simulink library "ammclib_bam_S32K3xx"  (R2016a)
(part 40 of 50)

      |       SampleTime=SampleTime_1;
      |       if isnan(SampleTime)
      |         hintText.Prompt='Note: Implementation parameters cannot be calculated yet because the block''s inherited sample time is unknown. Simulink will update the sample time when you run the simulation.';
      |       else
      |         hintText.Prompt='Caution: Implementation parameters depend on inherited sample time. Make sure that the sample time of the block''s inputs corresponds to the sampling period in the target application.';
      |       end
      |     else
      |       hintText.Prompt='Caution: Implementation parameters depend on the sample time. Make sure that the simulation time step corresponds to the sampling period in the target application.';
      |     end
      |     fltUpperLimit_bkup=get_param(gcb,'fltUpperLimit');
      |     fltLowerLimit_bkup=get_param(gcb,'fltLowerLimit');
      |     fltCC1sc_bkup=get_param(gcb,'fltCC1sc');
      |     fltCC2sc_bkup=get_param(gcb,'fltCC2sc');
      |     intmethod=get_param(gcb,'intmethod');
      |     pgain=Simulink.data.evalinGlobal(bdroot,get_param(gcb,'pgain'));
      |     igain=Simulink.data.evalinGlobal(bdroot,get_param(gcb,'igain'));
      |     upperLimit=Simulink.data.evalinGlobal(bdroot,get_param(gcb,'upperLimit'));
      |     lowerLimit=Simulink.data.evalinGlobal(bdroot,get_param(gcb,'lowerLimit'));
      |     if (upperLimit<=lowerLimit)
      |       warning('UpperLimit should be greater than LowerLimit.');
      |     end
      |     if strcmp(intmethod,'Forward Rectangular')
      |       cc1=pgain;
      |       cc2=-pgain+igain*SampleTime;
      |     else
      |       if strcmp(intmethod,'Backward Rectangular')
      |         cc1=pgain+igain*SampleTime;
      |         cc2=-pgain;
      |       else
      |         cc1=pgain+igain*SampleTime*0.5;
      |         cc2=-pgain+igain*SampleTime*0.5;
      |       end
      |     end
      |     fltCC1sc=cc1;
      |     fltCC2sc=cc2;
      |     fltUpperLimit=upperLimit;
      |     fltLowerLimit=lowerLimit;
      |     if isnan(fltUpperLimit)
      |       if ~strcmp(fltUpperLimit_bkup,'0')
      |         set_param(gcb,'fltUpperLimit','0');
      |       end
      |     else
      |       tmps=num2str(fltUpperLimit);
      |       if ~strcmp(fltUpperLimit_bkup,tmps)
      |         set_param(gcb,'fltUpperLimit',tmps);
      |       end
      |     end
      |     if isnan(fltLowerLimit)
      |       if ~strcmp(fltLowerLimit_bkup,'0')
      |         set_param(gcb,'fltLowerLimit','0');
      |       end
      |     else
      |       tmps=num2str(fltLowerLimit);
      |       if ~strcmp(fltLowerLimit_bkup,tmps)
      |         set_param(gcb,'fltLowerLimit',tmps);
      |       end
      |     end
      |     if isnan(fltCC1sc)
      |       if ~strcmp(fltCC1sc_bkup,'0')
      |         set_param(gcb,'fltCC1sc','0');
      |       end
      |     else
      |       tmps=num2str(fltCC1sc);
      |       if ~strcmp(fltCC1sc_bkup,tmps)
      |         set_param(gcb,'fltCC1sc',tmps);
      |       end
      |     end
      |     if isnan(fltCC2sc)
      |       if ~strcmp(fltCC2sc_bkup,'0')
      |         set_param(gcb,'fltCC2sc','0');
      |       end
      |     else
      |       tmps=num2str(fltCC2sc);
      |       if ~strcmp(fltCC2sc_bkup,tmps)
      |         set_param(gcb,'fltCC2sc',tmps);
      |       end
      |     end
      |   end
      | end
      mask TypeOptions intmethod: Forward Rectangular | Backward Rectangular | Trapezoidal
      mask Callback intmethod:
      | autoCalcEn=get_param(gcb,'autoCalcEn');
      | if strcmp(autoCalcEn,'on')
      |   SampleTime=Simulink.data.evalinGlobal(bdroot,get_param(gcb,'SampleTime'));
      |   if (SampleTime==-1)
      |     SampleTime=str2double(get_param(gcb,'SampleTime_1'));
      |   end
      |   fltUpperLimit_bkup=get_param(gcb,'fltUpperLimit');
      |   fltLowerLimit_bkup=get_param(gcb,'fltLowerLimit');
      |   fltCC1sc_bkup=get_param(gcb,'fltCC1sc');
      |   fltCC2sc_bkup=get_param(gcb,'fltCC2sc');
      |   intmethod=get_param(gcb,'intmethod');
      |   pgain=Simulink.data.evalinGlobal(bdroot,get_param(gcb,'pgain'));
      |   igain=Simulink.data.evalinGlobal(bdroot,get_param(gcb,'igain'));
      |   upperLimit=Simulink.data.evalinGlobal(bdroot,get_param(gcb,'upperLimit'));
      |   lowerLimit=Simulink.data.evalinGlobal(bdroot,get_param(gcb,'lowerLimit'));
      |   if (upperLimit<=lowerLimit)
      |     warning('UpperLimit should be greater than LowerLimit.');
      |   end
      |   if strcmp(intmethod,'Forward Rectangular')
      |     cc1=pgain;
      |     cc2=-pgain+igain*SampleTime;
      |   else
      |     if strcmp(intmethod,'Backward Rectangular')
      |       cc1=pgain+igain*SampleTime;
      |       cc2=-pgain;
      |     else
      |       cc1=pgain+igain*SampleTime*0.5;
      |       cc2=-pgain+igain*SampleTime*0.5;
      |     end
      |   end
      |   fltCC1sc=cc1;
      |   fltCC2sc=cc2;
      |   fltUpperLimit=upperLimit;
      |   fltLowerLimit=lowerLimit;
      |   if isnan(fltUpperLimit)
      |     if ~strcmp(fltUpperLimit_bkup,'0')
      |       set_param(gcb,'fltUpperLimit','0');
      |     end
      |   else
      |     tmps=num2str(fltUpperLimit);
      |     if ~strcmp(fltUpperLimit_bkup,tmps)
      |       set_param(gcb,'fltUpperLimit',tmps);
      |     end
      |   end
      |   if isnan(fltLowerLimit)
      |     if ~strcmp(fltLowerLimit_bkup,'0')
      |       set_param(gcb,'fltLowerLimit','0');
      |     end
      |   else
      |     tmps=num2str(fltLowerLimit);
      |     if ~strcmp(fltLowerLimit_bkup,tmps)
      |       set_param(gcb,'fltLowerLimit',tmps);
      |     end
      |   end
      |   if isnan(fltCC1sc)
      |     if ~strcmp(fltCC1sc_bkup,'0')
      |       set_param(gcb,'fltCC1sc','0');
      |     end
      |   else
      |     tmps=num2str(fltCC1sc);
      |     if ~strcmp(fltCC1sc_bkup,tmps)
      |       set_param(gcb,'fltCC1sc',tmps);
      |     end
      |   end
      |   if isnan(fltCC2sc)
      |     if ~strcmp(fltCC2sc_bkup,'0')
      |       set_param(gcb,'fltCC2sc','0');
      |     end
      |   else
      |     tmps=num2str(fltCC2sc);
      |     if ~strcmp(fltCC2sc_bkup,tmps)
      |       set_param(gcb,'fltCC2sc',tmps);
      |     end
      |   end
      | end
      mask Callback pgain:
      | autoCalcEn=get_param(gcb,'autoCalcEn');
      | if strcmp(autoCalcEn,'on')
      |   SampleTime=Simulink.data.evalinGlobal(bdroot,get_param(gcb,'SampleTime'));
      |   if (SampleTime==-1)
      |     SampleTime=str2double(get_param(gcb,'SampleTime_1'));
      |   end
      |   fltUpperLimit_bkup=get_param(gcb,'fltUpperLimit');
      |   fltLowerLimit_bkup=get_param(gcb,'fltLowerLimit');
      |   fltCC1sc_bkup=get_param(gcb,'fltCC1sc');
      |   fltCC2sc_bkup=get_param(gcb,'fltCC2sc');
      |   intmethod=get_param(gcb,'intmethod');
      |   pgain=Simulink.data.evalinGlobal(bdroot,get_param(gcb,'pgain'));
      |   igain=Simulink.data.evalinGlobal(bdroot,get_param(gcb,'igain'));
      |   upperLimit=Simulink.data.evalinGlobal(bdroot,get_param(gcb,'upperLimit'));
      |   lowerLimit=Simulink.data.evalinGlobal(bdroot,get_param(gcb,'lowerLimit'));
      |   if (upperLimit<=lowerLimit)
      |     warning('UpperLimit should be greater than LowerLimit.');
      |   end
      |   if strcmp(intmethod,'Forward Rectangular')
      |     cc1=pgain;
      |     cc2=-pgain+igain*SampleTime;
      |   else
      |     if strcmp(intmethod,'Backward Rectangular')
      |       cc1=pgain+igain*SampleTime;
      |       cc2=-pgain;
      |     else
      |       cc1=pgain+igain*SampleTime*0.5;
      |       cc2=-pgain+igain*SampleTime*0.5;
      |     end
      |   end
      |   fltCC1sc=cc1;
      |   fltCC2sc=cc2;
      |   fltUpperLimit=upperLimit;
      |   fltLowerLimit=lowerLimit;
      |   if isnan(fltUpperLimit)
      |     if ~strcmp(fltUpperLimit_bkup,'0')
      |       set_param(gcb,'fltUpperLimit','0');
      |     end
      |   else
      |     tmps=num2str(fltUpperLimit);
      |     if ~strcmp(fltUpperLimit_bkup,tmps)
      |       set_param(gcb,'fltUpperLimit',tmps);
      |     end
      |   end
      |   if isnan(fltLowerLimit)
      |     if ~strcmp(fltLowerLimit_bkup,'0')
      |       set_param(gcb,'fltLowerLimit','0');
      |     end
      |   else
      |     tmps=num2str(fltLowerLimit);
      |     if ~strcmp(fltLowerLimit_bkup,tmps)
      |       set_param(gcb,'fltLowerLimit',tmps);
      |     end
      |   end
      |   if isnan(fltCC1sc)
      |     if ~strcmp(fltCC1sc_bkup,'0')
      |       set_param(gcb,'fltCC1sc','0');
      |     end
      |   else
      |     tmps=num2str(fltCC1sc);
      |     if ~strcmp(fltCC1sc_bkup,tmps)
      |       set_param(gcb,'fltCC1sc',tmps);
      |     end
      |   end
      |   if isnan(fltCC2sc)
      |     if ~strcmp(fltCC2sc_bkup,'0')
      |       set_param(gcb,'fltCC2sc','0');
      |     end
      |   else
      |     tmps=num2str(fltCC2sc);
      |     if ~strcmp(fltCC2sc_bkup,tmps)
      |       set_param(gcb,'fltCC2sc',tmps);
      |     end
      |   end
      | end
      mask Callback igain:
      | autoCalcEn=get_param(gcb,'autoCalcEn');
      | if strcmp(autoCalcEn,'on')
      |   SampleTime=Simulink.data.evalinGlobal(bdroot,get_param(gcb,'SampleTime'));
      |   if (SampleTime==-1)
      |     SampleTime=str2double(get_param(gcb,'SampleTime_1'));
      |   end
      |   fltUpperLimit_bkup=get_param(gcb,'fltUpperLimit');
      |   fltLowerLimit_bkup=get_param(gcb,'fltLowerLimit');
      |   fltCC1sc_bkup=get_param(gcb,'fltCC1sc');
      |   fltCC2sc_bkup=get_param(gcb,'fltCC2sc');
      |   intmethod=get_param(gcb,'intmethod');
      |   pgain=Simulink.data.evalinGlobal(bdroot,get_param(gcb,'pgain'));
      |   igain=Simulink.data.evalinGlobal(bdroot,get_param(gcb,'igain'));
      |   upperLimit=Simulink.data.evalinGlobal(bdroot,get_param(gcb,'upperLimit'));
      |   lowerLimit=Simulink.data.evalinGlobal(bdroot,get_param(gcb,'lowerLimit'));
      |   if (upperLimit<=lowerLimit)
      |     warning('UpperLimit should be greater than LowerLimit.');
      |   end
      |   if strcmp(intmethod,'Forward Rectangular')
      |     cc1=pgain;
      |     cc2=-pgain+igain*SampleTime;
      |   else
      |     if strcmp(intmethod,'Backward Rectangular')
      |       cc1=pgain+igain*SampleTime;
      |       cc2=-pgain;
      |     else
      |       cc1=pgain+igain*SampleTime*0.5;
      |       cc2=-pgain+igain*SampleTime*0.5;
      |     end
      |   end
      |   fltCC1sc=cc1;
      |   fltCC2sc=cc2;
      |   fltUpperLimit=upperLimit;
      |   fltLowerLimit=lowerLimit;
      |   if isnan(fltUpperLimit)
      |     if ~strcmp(fltUpperLimit_bkup,'0')
      |       set_param(gcb,'fltUpperLimit','0');
      |     end
      |   else
      |     tmps=num2str(fltUpperLimit);
      |     if ~strcmp(fltUpperLimit_bkup,tmps)
      |       set_param(gcb,'fltUpperLimit',tmps);
      |     end
      |   end
      |   if isnan(fltLowerLimit)
      |     if ~strcmp(fltLowerLimit_bkup,'0')
      |       set_param(gcb,'fltLowerLimit','0');
      |     end
      |   else
      |     tmps=num2str(fltLowerLimit);
      |     if ~strcmp(fltLowerLimit_bkup,tmps)
      |       set_param(gcb,'fltLowerLimit',tmps);
      |     end
      |   end
      |   if isnan(fltCC1sc)
      |     if ~strcmp(fltCC1sc_bkup,'0')
      |       set_param(gcb,'fltCC1sc','0');
      |     end
      |   else
      |     tmps=num2str(fltCC1sc);
      |     if ~strcmp(fltCC1sc_bkup,tmps)
      |       set_param(gcb,'fltCC1sc',tmps);
      |     end
      |   end
      |   if isnan(fltCC2sc)
      |     if ~strcmp(fltCC2sc_bkup,'0')
      |       set_param(gcb,'fltCC2sc','0');
      |     end
      |   else
      |     tmps=num2str(fltCC2sc);
      |     if ~strcmp(fltCC2sc_bkup,tmps)
      |       set_param(gcb,'fltCC2sc',tmps);
      |     end
      |   end
      | end
      mask Callback upperLimit:
      | autoCalcEn=get_param(gcb,'autoCalcEn');
      | if strcmp(autoCalcEn,'on')
      |   SampleTime=Simulink.data.evalinGlobal(bdroot,get_param(gcb,'SampleTime'));
      |   if (SampleTime==-1)
      |     SampleTime=str2double(get_param(gcb,'SampleTime_1'));
      |   end
      |   fltUpperLimit_bkup=get_param(gcb,'fltUpperLimit');
      |   fltLowerLimit_bkup=get_param(gcb,'fltLowerLimit');
      |   fltCC1sc_bkup=get_param(gcb,'fltCC1sc');
      |   fltCC2sc_bkup=get_param(gcb,'fltCC2sc');
      |   intmethod=get_param(gcb,'intmethod');
      |   pgain=Simulink.data.evalinGlobal(bdroot,get_param(gcb,'pgain'));
      |   igain=Simulink.data.evalinGlobal(bdroot,get_param(gcb,'igain'));
      |   upperLimit=Simulink.data.evalinGlobal(bdroot,get_param(gcb,'upperLimit'));
      |   lowerLimit=Simulink.data.evalinGlobal(bdroot,get_param(gcb,'lowerLimit'));
      |   if (upperLimit<=lowerLimit)
      |     warning('UpperLimit should be greater than LowerLimit.');
      |   end
      |   if strcmp(intmethod,'Forward Rectangular')
      |     cc1=pgain;
      |     cc2=-pgain+igain*SampleTime;
      |   else
      |     if strcmp(intmethod,'Backward Rectangular')
      |       cc1=pgain+igain*SampleTime;
      |       cc2=-pgain;
      |     else
      |       cc1=pgain+igain*SampleTime*0.5;
      |       cc2=-pgain+igain*SampleTime*0.5;
      |     end
      |   end
      |   fltCC1sc=cc1;
      |   fltCC2sc=cc2;
      |   fltUpperLimit=upperLimit;
      |   fltLowerLimit=lowerLimit;
      |   if isnan(fltUpperLimit)
      |     if ~strcmp(fltUpperLimit_bkup,'0')
      |       set_param(gcb,'fltUpperLimit','0');
      |     end
      |   else
      |     tmps=num2str(fltUpperLimit);
      |     if ~strcmp(fltUpperLimit_bkup,tmps)
      |       set_param(gcb,'fltUpperLimit',tmps);
      |     end
      |   end
      |   if isnan(fltLowerLimit)
      |     if ~strcmp(fltLowerLimit_bkup,'0')
      |       set_param(gcb,'fltLowerLimit','0');
      |     end
      |   else
      |     tmps=num2str(fltLowerLimit);
      |     if ~strcmp(fltLowerLimit_bkup,tmps)
      |       set_param(gcb,'fltLowerLimit',tmps);
      |     end
      |   end
      |   if isnan(fltCC1sc)
      |     if ~strcmp(fltCC1sc_bkup,'0')
      |       set_param(gcb,'fltCC1sc','0');
      |     end
      |   else
      |     tmps=num2str(fltCC1sc);
      |     if ~strcmp(fltCC1sc_bkup,tmps)
      |       set_param(gcb,'fltCC1sc',tmps);
      |     end
      |   end
      |   if isnan(fltCC2sc)
      |     if ~strcmp(fltCC2sc_bkup,'0')
      |       set_param(gcb,'fltCC2sc','0');
      |     end
      |   else
      |     tmps=num2str(fltCC2sc);
      |     if ~strcmp(fltCC2sc_bkup,tmps)
      |       set_param(gcb,'fltCC2sc',tmps);
      |     end
      |   end
      | end
      mask Callback lowerLimit:
      | autoCalcEn=get_param(gcb,'autoCalcEn');
      | if strcmp(autoCalcEn,'on')
      |   SampleTime=Simulink.data.evalinGlobal(bdroot,get_param(gcb,'SampleTime'));
      |   if (SampleTime==-1)
      |     SampleTime=str2double(get_param(gcb,'SampleTime_1'));
      |   end
      |   fltUpperLimit_bkup=get_param(gcb,'fltUpperLimit');
      |   fltLowerLimit_bkup=get_param(gcb,'fltLowerLimit');
      |   fltCC1sc_bkup=get_param(gcb,'fltCC1sc');
      |   fltCC2sc_bkup=get_param(gcb,'fltCC2sc');
      |   intmethod=get_param(gcb,'intmethod');
      |   pgain=Simulink.data.evalinGlobal(bdroot,get_param(gcb,'pgain'));
      |   igain=Simulink.data.evalinGlobal(bdroot,get_param(gcb,'igain'));
      |   upperLimit=Simulink.data.evalinGlobal(bdroot,get_param(gcb,'upperLimit'));
      |   lowerLimit=Simulink.data.evalinGlobal(bdroot,get_param(gcb,'lowerLimit'));
      |   if (upperLimit<=lowerLimit)
      |     warning('UpperLimit should be greater than LowerLimit.');
      |   end
      |   if strcmp(intmethod,'Forward Rectangular')
      |     cc1=pgain;
      |     cc2=-pgain+igain*SampleTime;
      |   else
      |     if strcmp(intmethod,'Backward Rectangular')
      |       cc1=pgain+igain*SampleTime;
      |       cc2=-pgain;
      |     else
      |       cc1=pgain+igain*SampleTime*0.5;
      |       cc2=-pgain+igain*SampleTime*0.5;
      |     end
      |   end
      |   fltCC1sc=cc1;
      |   fltCC2sc=cc2;
      |   fltUpperLimit=upperLimit;
      |   fltLowerLimit=lowerLimit;
      |   if isnan(fltUpperLimit)
      |     if ~strcmp(fltUpperLimit_bkup,'0')
      |       set_param(gcb,'fltUpperLimit','0');
      |     end
      |   else
      |     tmps=num2str(fltUpperLimit);
      |     if ~strcmp(fltUpperLimit_bkup,tmps)
      |       set_param(gcb,'fltUpperLimit',tmps);
      |     end
      |   end
      |   if isnan(fltLowerLimit)
      |     if ~strcmp(fltLowerLimit_bkup,'0')
      |       set_param(gcb,'fltLowerLimit','0');
      |     end
      |   else
      |     tmps=num2str(fltLowerLimit);
      |     if ~strcmp(fltLowerLimit_bkup,tmps)
      |       set_param(gcb,'fltLowerLimit',tmps);
      |     end
      |   end
      |   if isnan(fltCC1sc)
      |     if ~strcmp(fltCC1sc_bkup,'0')
      |       set_param(gcb,'fltCC1sc','0');
      |     end
      |   else
      |     tmps=num2str(fltCC1sc);
      |     if ~strcmp(fltCC1sc_bkup,tmps)
      |       set_param(gcb,'fltCC1sc',tmps);
      |     end
      |   end
      |   if isnan(fltCC2sc)
      |     if ~strcmp(fltCC2sc_bkup,'0')
      |       set_param(gcb,'fltCC2sc','0');
      |     end
      |   else
      |     tmps=num2str(fltCC2sc);
      |     if ~strcmp(fltCC2sc_bkup,tmps)
      |       set_param(gcb,'fltCC2sc',tmps);
      |     end
      |   end
      | end
      mask Callback autoCalcEn:
      | maskStr=get_param(gcb,'showStates');
      | if strcmp(maskStr,'Hide (faster execution)')
      |   p=Simulink.Mask.get(gcb);
      |   autoCalcEn=get_param(gcb,'autoCalcEn');
      |   hintText=p.getDialogControl('timeHint');
      |   if strcmp(autoCalcEn,'on')
      |     param=p.getParameter('lowerLimit');
      |     if strcmp(param.Enabled,'off')
      |       SampleTime=Simulink.data.evalinGlobal(bdroot,get_param(gcb,'SampleTime'));
      |       if SampleTime==-1
      |         SampleTime=str2double(get_param(gcb,'SampleTime_1'));
      |         if isnan(SampleTime)
      |           hintText.Prompt=['Note: Implementation parameters cannot be calculated yet because the block''s inherited sample time is unknown. Simulink will update the sample time when you run the simulation.'];
      |         else
      |           hintText.Prompt=['Caution: Implementation parameters depend on inherited sample time. Make sure that the sample time of the block''s inputs corresponds to the sampling period in the target application.'];
      |         end
      |       else
      |         hintText.Prompt='Caution: Implementation parameters depend on the sample time. Make sure that the simulation time step corresponds to the sampling period in the target application.';
      |       end
      |       p=Simulink.Mask.get(gcb);
      |       param=p.getParameter('intmethod');
      |       param.set('Enabled','on');
      |       param=p.getParameter('pgain');
      |       param.set('Enabled','on');
      |       param=p.getParameter('igain');
      |       param.set('Enabled','on');
      |       param=p.getParameter('upperLimit');
      |       param.set('Enabled','on');
      |       param=p.getParameter('lowerLimit');
      |       param.set('Enabled','on');
      |     else
      |       SampleTime=Simulink.data.evalinGlobal(bdroot,get_param(gcb,'SampleTime'));
      |       if SampleTime==-1
      |         SampleTime=str2double(get_param(gcb,'SampleTime_1'));
      |       end
      |     end
      |     fltUpperLimit_bkup=get_param(gcb,'fltUpperLimit');
      |     fltLowerLimit_bkup=get_param(gcb,'fltLowerLimit');
      |     fltCC1sc_bkup=get_param(gcb,'fltCC1sc');
      |     fltCC2sc_bkup=get_param(gcb,'fltCC2sc');
      |     intmethod=get_param(gcb,'intmethod');
      |     pgain=Simulink.data.evalinGlobal(bdroot,get_param(gcb,'pgain'));
      |     igain=Simulink.data.evalinGlobal(bdroot,get_param(gcb,'igain'));
      |     upperLimit=Simulink.data.evalinGlobal(bdroot,get_param(gcb,'upperLimit'));
      |     lowerLimit=Simulink.data.evalinGlobal(bdroot,get_param(gcb,'lowerLimit'));
      |     if (upperLimit<=lowerLimit)
      |       warning('UpperLimit should be greater than LowerLimit.');
      |     end
      |     if strcmp(intmethod,'Forward Rectangular')
      |       cc1=pgain;
      |       cc2=-pgain+igain*SampleTime;
      |     else
      |       if strcmp(intmethod,'Backward Rectangular')
      |         cc1=pgain+igain*SampleTime;
      |         cc2=-pgain;
      |       else
      |         cc1=pgain+igain*SampleTime*0.5;
      |         cc2=-pgain+igain*SampleTime*0.5;
      |       end
      |     end
      |     fltCC1sc=cc1;
      |     fltCC2sc=cc2;
      |     fltUpperLimit=upperLimit;
      |     fltLowerLimit=lowerLimit;
      |     if isnan(fltUpperLimit)
      |       if ~strcmp(fltUpperLimit_bkup,'0')
      |         set_param(gcb,'fltUpperLimit','0');
      |       end
      |     else
      |       tmps=num2str(fltUpperLimit);
      |       if ~strcmp(fltUpperLimit_bkup,tmps)
      |         set_param(gcb,'fltUpperLimit',tmps);
      |       end
      |     end
      |     if isnan(fltLowerLimit)
      |       if ~strcmp(fltLowerLimit_bkup,'0')
      |         set_param(gcb,'fltLowerLimit','0');
      |       end
      |     else
      |       tmps=num2str(fltLowerLimit);
      |       if ~strcmp(fltLowerLimit_bkup,tmps)
      |         set_param(gcb,'fltLowerLimit',tmps);
      |       end
      |     end
      |     if isnan(fltCC1sc)
      |       if ~strcmp(fltCC1sc_bkup,'0')
      |         set_param(gcb,'fltCC1sc','0');
      |       end
      |     else
      |       tmps=num2str(fltCC1sc);
      |       if ~strcmp(fltCC1sc_bkup,tmps)
      |         set_param(gcb,'fltCC1sc',tmps);
      |       end
      |     end
      |     if isnan(fltCC2sc)
      |       if ~strcmp(fltCC2sc_bkup,'0')
      |         set_param(gcb,'fltCC2sc','0');
      |       end
      |     else
      |       tmps=num2str(fltCC2sc);
      |       if ~strcmp(fltCC2sc_bkup,tmps)
      |         set_param(gcb,'fltCC2sc',tmps);
      |       end
      |     end
      |   else
      |     param=p.getParameter('lowerLimit');
      |     if strcmp(param.Enabled,'on')
      |       hintText.Prompt='Caution: Implementation parameters are fixed.';
      |       p=Simulink.Mask.get(gcb);
      |       param=p.getParameter('intmethod');
      |       param.set('Enabled','off');
      |       param=p.getParameter('pgain');
      |       param.set('Enabled','off');
      |       param=p.getParameter('igain');
      |       param.set('Enabled','off');
      |       param=p.getParameter('upperLimit');
      |       param.set('Enabled','off');
      |       param=p.getParameter('lowerLimit');
      |       param.set('Enabled','off');
      |     end
      |   end
      | end
      mask DialogControl CompBut Prompt: Recalculate sample times
      mask DialogControl CompBut Tooltip: Simulink updates the sample times of all blocks when the simulation is run. This button will update the sample times now.
      mask DialogControl CompBut Callback:
      | btn=questdlg('This will apply all changes in all open dialog boxes and update the schematic. Do you want to proceed?','Apply all changes','Continue','Cancel','Continue');
      | if strcmp(btn,'Continue')
      |   dlgs=DAStudio.ToolRoot.getOpenDialogs;
      |   for i=1:length(dlgs)
      |     dlgs(i).apply;
      |   end
      |   try
      |     SampleTime_1=str2double(get_param(gcb,'SampleTime_1'));
      |     ts=Simulink.Block.getSampleTimes(gcb);
      |     ts=ts(1).Value(1);
      |     if (SampleTime_1 ~= ts)
      |       SampleTime_1=ts;
      |       set_param(gcb,'SampleTime_1',num2str(ts));
      |       autoCalcEn=get_param(gcb,'autoCalcEn');
      |       if strcmp(autoCalcEn,'on')
      |         SampleTime=Simulink.data.evalinGlobal(bdroot,get_param(gcb,'SampleTime'));
      |         p=Simulink.Mask.get(gcb);
      |         hintText=p.getDialogControl('timeHint');
      |         if SampleTime==-1
      |           SampleTime=SampleTime_1;
      |           hintText.Prompt='Caution: Implementation parameters depend on inherited sample time. Make sure that the sample time of the block''s inputs corresponds to the sampling period in the target application.';
      |         else
      |           hintText.Prompt='Caution: Implementation parameters depend on the sample time. Make sure that the simulation time step corresponds to the sampling period in the target application.';
      |         end
      |         fltUpperLimit_bkup=get_param(gcb,'fltUpperLimit');
      |         fltLowerLimit_bkup=get_param(gcb,'fltLowerLimit');
      |         fltCC1sc_bkup=get_param(gcb,'fltCC1sc');
      |         fltCC2sc_bkup=get_param(gcb,'fltCC2sc');
      |         intmethod=get_param(gcb,'intmethod');
      |         pgain=Simulink.data.evalinGlobal(bdroot,get_param(gcb,'pgain'));
      |         igain=Simulink.data.evalinGlobal(bdroot,get_param(gcb,'igain'));
      |         upperLimit=Simulink.data.evalinGlobal(bdroot,get_param(gcb,'upperLimit'));
      |         lowerLimit=Simulink.data.evalinGlobal(bdroot,get_param(gcb,'lowerLimit'));
      |         if (upperLimit<=lowerLimit)
      |           warning('UpperLimit should be greater than LowerLimit.');
      |         end
      |         if strcmp(intmethod,'Forward Rectangular')
      |           cc1=pgain;
      |           cc2=-pgain+igain*SampleTime;
      |         else
      |           if strcmp(intmethod,'Backward Rectangular')
      |             cc1=pgain+igain*SampleTime;
      |             cc2=-pgain;
      |           else
      |             cc1=pgain+igain*SampleTime*0.5;
      |             cc2=-pgain+igain*SampleTime*0.5;
      |           end
      |         end
      |         fltCC1sc=cc1;
      |         fltCC2sc=cc2;
      |         fltUpperLimit=upperLimit;
      |         fltLowerLimit=lowerLimit;
      |         if isnan(fltUpperLimit)
      |           if ~strcmp(fltUpperLimit_bkup,'0')
      |             set_param(gcb,'fltUpperLimit','0');
      |           end
      |         else
      |           tmps=num2str(fltUpperLimit);
      |           if ~strcmp(fltUpperLimit_bkup,tmps)
      |             set_param(gcb,'fltUpperLimit',tmps);
      |           end
      |         end
      |         if isnan(fltLowerLimit)
      |           if ~strcmp(fltLowerLimit_bkup,'0')
      |             set_param(gcb,'fltLowerLimit','0');
      |           end
      |         else
      |           tmps=num2str(fltLowerLimit);
      |           if ~strcmp(fltLowerLimit_bkup,tmps)
      |             set_param(gcb,'fltLowerLimit',tmps);
      |           end
      |         end
      |         if isnan(fltCC1sc)
      |           if ~strcmp(fltCC1sc_bkup,'0')
      |             set_param(gcb,'fltCC1sc','0');
      |           end
      |         else
      |           tmps=num2str(fltCC1sc);
      |           if ~strcmp(fltCC1sc_bkup,tmps)
      |             set_param(gcb,'fltCC1sc',tmps);
      |           end
      |         end
      |         if isnan(fltCC2sc)
      |           if ~strcmp(fltCC2sc_bkup,'0')
      |             set_param(gcb,'fltCC2sc','0');
      |           end
      |         else
      |           tmps=num2str(fltCC2sc);
      |           if ~strcmp(fltCC2sc_bkup,tmps)
      |             set_param(gcb,'fltCC2sc',tmps);
      |           end
      |         end
      |       end
      |     end
      |   catch
      |    warning(['Sample time cannot be calculated for the block ' gcb])
      |   end
      | end
      mask DialogControl timeHint Prompt: Note: Implementation parameters cannot be calculated yet because the block's inherited sample time is unknown. Simulink will update the sample time when you run the simulation.
      mask Display:
      | color('black');
      | pos = get_param(gcb, 'Position');
      | width = pos(3) - pos(1);
      | height = pos(4) - pos(2);
      | tX=width/2;
      | tY=height - 25;
      | color('black');
      | text(tX,tY, 'GFLIB_ControllerPIrAW_FLT', 'horizontalAlignment', 'center');
      | if showStates == 2
      |   color('red');
      |   text(tX,tY - 20, ['debugging mode' char(13) char(10) '(limited performance)'], 'horizontalAlignment', 'center');
      | end
  GFLIB_ControllerPIr_FLT : Subsystem  StartFcn=|  TreatAsAtomicUnit=on  mask(GFLIB_ControllerPIr_FLT){showStates=Hide (faster execution), resetStatesEnable=Pre-set according to the first set of inputs after reset, SampleTime=-1, intmethod=Trapezoidal, pgain=5, igain=0.5, autoCalcEn=on, fltCC1sc=0, fltCC2sc=0, SampleTime_1=NaN}
      | ts=get_param(gcb,'CompiledSampleTime');
      | if iscell(ts)
      |   ts=ts{1};
      |   if iscell(ts)
      |     ts=ts{1};
      |   end
      | end
      | ts=ts(1);
      | set_param(gcb,'SampleTime_1',num2str(ts));
      | p=Simulink.Mask.get(gcb);
      | hintText=p.getDialogControl('timeHint');
      | SampleTime=Simulink.data.evalinGlobal(bdroot,get_param(gcb,'SampleTime'));
      | p=Simulink.Mask.get(gcb);
      | autoCalcEn=get_param(gcb,'autoCalcEn');
      | if strcmp(autoCalcEn,'on')
      |   if SampleTime==-1
      |     hintText.Prompt='Caution: Implementation parameters depend on inherited sample time. Make sure that the sample time of the block''s inputs corresponds to the sampling period in the target application.';
      |   else
      |     hintText.Prompt='Caution: Implementation parameters depend on the sample time. Make sure that the simulation time step corresponds to the sampling period in the target application.';
      |   end
      |   SampleTime=ts;
      |   fltCC1sc_bkup=get_param(gcb,'fltCC1sc');
      |   fltCC2sc_bkup=get_param(gcb,'fltCC2sc');
      |   intmethod=get_param(gcb,'intmethod');
      |   pgain=Simulink.data.evalinGlobal(bdroot,get_param(gcb,'pgain'));
      |   igain=Simulink.data.evalinGlobal(bdroot,get_param(gcb,'igain'));
      |   if strcmp(intmethod,'Forward Rectangular')
      |     cc1=pgain;
      |     cc2=-pgain+igain*SampleTime;
      |   else
      |     if strcmp(intmethod,'Backward Rectangular')
      |       cc1=pgain+igain*SampleTime;
      |       cc2=-pgain;
      |     else
      |       cc1=pgain+igain*SampleTime*0.5;
      |       cc2=-pgain+igain*SampleTime*0.5;
      |     end
      |   end
      |   fltCC1sc=cc1;
      |   fltCC2sc=cc2;
      |   if isnan(fltCC1sc)
      |     if ~strcmp(fltCC1sc_bkup,'0')
      |       set_param(gcb,'fltCC1sc','0');
      |     end
      |   else
      |     tmps=num2str(fltCC1sc);
      |     if ~strcmp(fltCC1sc_bkup,tmps)
      |       set_param(gcb,'fltCC1sc',tmps);
      |     end
      |   end
      |   if isnan(fltCC2sc)
      |     if ~strcmp(fltCC2sc_bkup,'0')
      |       set_param(gcb,'fltCC2sc','0');
      |     end
      |   else
      |     tmps=num2str(fltCC2sc);
      |     if ~strcmp(fltCC2sc_bkup,tmps)
      |       set_param(gcb,'fltCC2sc',tmps);
      |     end
      |   end
      | end
      mask prompts: showStates "Show internal states:"; resetStatesEnable "Internal state after reset:"; SampleTime "Sample time (-1 for inherited):"; intmethod "Integration method:"; pgain "Proportional gain (P):"; igain "Integral gain (I):"; autoCalcEn "Calculate implementation parameters from physical parameters"; fltCC1sc "fltCC1sc (CC1 coefficient):"; fltCC2sc "fltCC2sc (CC2 coefficient):"; SampleTime_1 "Discrete sample time:"
      mask help: Recurrent form discrete-time PI controller without anti-windup in single precision floating-point implementation. This block supports re-initialization of the internal state during simulation. If the block is reset, the controller's output will be aligned with the input fltControllerPIrOut_preset. Refer to the AMMCLIB User's Guide for further details.
      mask init:
      | ddName = get_param(bdroot,'DataDictionary');
      | if length(ddName)==0
      |   set_param(bdroot,'DataDictionary','ammclib_types.sldd');
      | else
      |   dd = Simulink.data.dictionary.open(ddName);
      |   data = getSection(dd,'Design Data');
      |   if ~exist(data,'SWLIBS_2Syst_F16')
      |     addDataSource(dd,'ammclib_types.sldd');
      |     saveChanges(dd);
      |   end
      | end
      | 
      | if showStates == 1
      |   % hidden state variables
      |   if strcmp(get_param([gcb '/fltCC1sc'], 'BlockType'), 'Inport')
      |     posblk = get_param(gcb, 'Position');
      | 
      |     pos = get_param([gcb, '/fltCC1sc'], 'Position');
      |     orient = get_param([gcb, '/fltCC1sc'], 'Orientation');
      |     delete_block([gcb, '/fltCC1sc']);
      |     add_block('built-in/Ground', [gcb, '/fltCC1sc'], 'Position', pos, 'Orientation', orient);
      | 
      |     pos = get_param([gcb, '/fltCC2sc'], 'Position');
      |     orient = get_param([gcb, '/fltCC2sc'], 'Orientation');
      |     delete_block([gcb, '/fltCC2sc']);
      |     add_block('built-in/Ground', [gcb, '/fltCC2sc'], 'Position', pos, 'Orientation', orient);
      | 
      |     pos = get_param([gcb, '/fltAcc'], 'Position');
      |     orient = get_param([gcb, '/fltAcc'], 'Orientation');
      |     delete_block([gcb, '/fltAcc']);
      |     add_block('built-in/Ground', [gcb, '/fltAcc'], 'Position', pos, 'Orientation', orient);
      | 
      |     pos = get_param([gcb, '/fltInErrK1'], 'Position');
      |     orient = get_param([gcb, '/fltInErrK1'], 'Orientation');
      |     delete_block([gcb, '/fltInErrK1']);
      |     add_block('built-in/Ground', [gcb, '/fltInErrK1'], 'Position', pos, 'Orientation', orient);
      | 
      | 
      |     pmask=Simulink.Mask.get(gcb);
      |     pctrl=pmask.getParameter('SampleTime');
      |     pctrl.set('TypeOptions',{'fltInErr/SampleTime','fltControllerPIrOut_preset/SampleTime'});
      | 
      |     pos = get_param([gcb '/fltAcc_Out'], 'Position');
      |     orient = get_param([gcb '/fltAcc_Out'], 'Orientation');
      |     delete_block([gcb '/fltAcc_Out']);
      |     add_block('built-in/Terminator', [gcb '/fltAcc_Out'], 'Position', pos, 'Orientation', orient);
      | 
      |     pos = get_param([gcb '/fltInErrK1_Out'], 'Position');
      |     orient = get_param([gcb '/fltInErrK1_Out'], 'Orientation');
      |     delete_block([gcb '/fltInErrK1_Out']);
      |     add_block('built-in/Terminator', [gcb '/fltInErrK1_Out'], 'Position', pos, 'Orientation', orient);
      | 
      |     set_param([gcb '/fltInErr'], 'Port', '1');
      |     set_param([gcb '/fltControllerPIrOut_preset'], 'Port', '2');
      | 
      |     tmpOutCnt=0;
      |     tmpOutCnt=tmpOutCnt+1;
      |     set_param([gcb '/fltOut'], 'Port', num2str(tmpOutCnt));
      | 
      |     autoCalcEn=get_param(gcb,'autoCalcEn');
      |     if strcmp(autoCalcEn,'on')
      |       set_param(gcb,'MaskEnables',{'on','on','on','on','on','on','on','on','on','off'});
      |     else
      |       set_param(gcb,'MaskEnables',{'on','on','on','off','off','off','on','on','on','off'});
      |     end
      | 
      |     if (posblk(4) - posblk(2)) > 75
      |       height = 75;
      |       set_param(gcb,'Position',[posblk(1), posblk(2), posblk(3), posblk(2)+height])
      |     end
      |   end
      | else
      |   % shown state variables
      |   if strcmp(get_param([gcb '/fltCC1sc'], 'BlockType'), 'Ground')
      |     posblk = get_param(gcb, 'Position');
      | 
      |     pos = get_param([gcb, '/fltCC1sc'], 'Position');
      |     orient = get_param([gcb, '/fltCC1sc'], 'Orientation');
      |     delete_block([gcb, '/fltCC1sc']);
      |     add_block('built-in/Inport', [gcb, '/fltCC1sc'], 'Position', pos, 'Orientation', orient, 'OutDataTypeStr', 'single');
      | 
      |     pos = get_param([gcb, '/fltCC2sc'], 'Position');
      |     orient = get_param([gcb, '/fltCC2sc'], 'Orientation');
      |     delete_block([gcb, '/fltCC2sc']);
      |     add_block('built-in/Inport', [gcb, '/fltCC2sc'], 'Position', pos, 'Orientation', orient, 'OutDataTypeStr', 'single');
      | 
      |     pos = get_param([gcb, '/fltAcc'], 'Position');
      |     orient = get_param([gcb, '/fltAcc'], 'Orientation');
      |     delete_block([gcb, '/fltAcc']);
      |     add_block('built-in/Inport', [gcb, '/fltAcc'], 'Position', pos, 'Orientation', orient, 'OutDataTypeStr', 'single');
      | 
      |     pos = get_param([gcb, '/fltInErrK1'], 'Position');
      |     orient = get_param([gcb, '/fltInErrK1'], 'Orientation');
      |     delete_block([gcb, '/fltInErrK1']);
      |     add_block('built-in/Inport', [gcb, '/fltInErrK1'], 'Position', pos, 'Orientation', orient, 'OutDataTypeStr', 'single');
      | 
      | 
      | 
      |     pos = get_param([gcb '/fltAcc_Out'], 'Position');
      |     orient = get_param([gcb '/fltAcc_Out'], 'Orientation');
      |     delete_block([gcb '/fltAcc_Out']);
      |     add_block('built-in/Outport', [gcb '/fltAcc_Out'], 'Position', pos, 'Orientation', orient);
      | 
      |     pos = get_param([gcb '/fltInErrK1_Out'], 'Position');
      |     orient = get_param([gcb '/fltInErrK1_Out'], 'Orientation');
      |     delete_block([gcb '/fltInErrK1_Out']);
      |     add_block('built-in/Outport', [gcb '/fltInErrK1_Out'], 'Position', pos, 'Orientation', orient);
      | 
      | 
      |     pmask=Simulink.Mask.get(gcb);
      |     pctrl=pmask.getParameter('SampleTime');
      |     pctrl.set('TypeOptions',{'fltInErr/SampleTime','fltControllerPIrOut_preset/SampleTime','fltCC1sc/SampleTime','fltCC2sc/SampleTime','fltAcc/SampleTime','fltInErrK1/SampleTime'});
      | 
      |     set_param([gcb '/fltInErr'], 'Port', '1');
      |     set_param([gcb '/fltControllerPIrOut_preset'], 'Port', '2');
      |     set_param([gcb '/fltCC1sc'], 'Port', '3');
      |     set_param([gcb '/fltCC2sc'], 'Port', '4');
      |     set_param([gcb '/fltAcc'], 'Port', '5');
      |     set_param([gcb '/fltInErrK1'], 'Port', '6');
      | 
      |     tmpOutCnt=0;
      |     tmpOutCnt=tmpOutCnt+1;
      |     set_param([gcb '/fltOut'], 'Port', num2str(tmpOutCnt));
      |     tmpOutCnt=tmpOutCnt+1;
      |     set_param([gcb '/fltAcc_Out'], 'Port', num2str(tmpOutCnt));
      |     tmpOutCnt=tmpOutCnt+1;
      |     set_param([gcb '/fltInErrK1_Out'], 'Port', num2str(tmpOutCnt));
      | 
      |     set_param(gcb,'MaskEnables',{'on','on','on','off','off','off','off','off','off','off'});
      | 
      |     if (posblk(4) - posblk(2)) < 175
      |       height = 175;
      |       set_param(gcb,'Position',[posblk(1), posblk(2), posblk(3), posblk(2)+height])
      |     end
      |   end
      | end
      settings: RTWSystemCode=Inline
      mask Help: web([fileparts(which('ammclib_bam_S32K3xx.slx')) '/../doc/S32K3XXMCLUG.pdf'], '-browser')
      mask TypeOptions showStates: Hide (faster execution) | Show (allows debugging; connect feedback loops manually)
      mask Callback showStates:
      | maskStr=get_param(gcb,'showStates');
      | if strcmp(maskStr,'Hide (faster execution)')
      |   if strcmp(get_param([gcb '/fltCC1sc'], 'BlockType'), 'Inport')
      |     autoCalcEn=get_param(gcb,'autoCalcEn');
      |     if strcmp(autoCalcEn,'on')
      |       set_param(gcb,'MaskEnables',{'on','on','on','on','on','on','on','on','on','off'});
      |     else
      |       set_param(gcb,'MaskEnables',{'on','on','on','off','off','off','on','on','on','off'});
      |     end
      |   end
      | else
      |   if strcmp(get_param([gcb '/fltCC1sc'], 'BlockType'), 'Ground')
      |     set_param(gcb,'MaskEnables',{'on','on','on','off','off','off','off','off','off','off'});
      |   end
      | end
      mask TypeOptions resetStatesEnable: Pre-set according to the first set of inputs after reset | Clear to zero
      mask TypeOptions SampleTime: fltInErr/SampleTime | fltControllerPIrOut_preset/SampleTime
      mask Callback SampleTime:
      | p=Simulink.Mask.get(gcb);
      | hintText=p.getDialogControl('timeHint');
      | SampleTime=Simulink.data.evalinGlobal(bdroot,get_param(gcb,'SampleTime'));
      | SampleTime_1=str2double(get_param(gcb,'SampleTime_1'));
      | if (((SampleTime==-1) && (~contains(hintText.Prompt,'inherited'))) || ...
      |     ((SampleTime~=-1) && contains(hintText.Prompt,'inherited')) || ...
      |     ((SampleTime~=-1) && (SampleTime_1~=SampleTime)) || ...
      |     ((SampleTime_1~=-1) && contains(hintText.Prompt,'yet')))
      |   if ((SampleTime==-1) && (~contains(hintText.Prompt,'inherited')))
      |     set_param(gcb,'SampleTime_1',num2str(NaN));
      |     SampleTime_1=NaN;
      |   end
      |   if (SampleTime~=-1)
      |     set_param(gcb,'SampleTime_1',num2str(SampleTime));
      |     SampleTime_1=SampleTime;
      |   end
      |   autoCalcEn=get_param(gcb,'autoCalcEn');
      |   if strcmp(autoCalcEn,'on')
      |     p=Simulink.Mask.get(gcb);
      |     hintText=p.getDialogControl('timeHint');
      |     if SampleTime==-1
      |       SampleTime=SampleTime_1;
      |       if isnan(SampleTime)
      |         hintText.Prompt='Note: Implementation parameters cannot be calculated yet because the block''s inherited sample time is unknown. Simulink will update the sample time when you run the simulation.';
      |       else
      |         hintText.Prompt='Caution: Implementation parameters depend on inherited sample time. Make sure that the sample time of the block''s inputs corresponds to the sampling period in the target application.';
      |       end
      |     else
      |       hintText.Prompt='Caution: Implementation parameters depend on the sample time. Make sure that the simulation time step corresponds to the sampling period in the target application.';
      |     end
      |     fltCC1sc_bkup=get_param(gcb,'fltCC1sc');
      |     fltCC2sc_bkup=get_param(gcb,'fltCC2sc');
      |     intmethod=get_param(gcb,'intmethod');
      |     pgain=Simulink.data.evalinGlobal(bdroot,get_param(gcb,'pgain'));
      |     igain=Simulink.data.evalinGlobal(bdroot,get_param(gcb,'igain'));
      |     if strcmp(intmethod,'Forward Rectangular')
      |       cc1=pgain;
      |       cc2=-pgain+igain*SampleTime;
      |     else
      |       if strcmp(intmethod,'Backward Rectangular')
      |         cc1=pgain+igain*SampleTime;
      |         cc2=-pgain;
      |       else
      |         cc1=pgain+igain*SampleTime*0.5;
      |         cc2=-pgain+igain*SampleTime*0.5;
      |       end
      |     end
      |     fltCC1sc=cc1;
      |     fltCC2sc=cc2;
      |     if isnan(fltCC1sc)
      |       if ~strcmp(fltCC1sc_bkup,'0')
      |         set_param(gcb,'fltCC1sc','0');
      |       end
      |     else
      |       tmps=num2str(fltCC1sc);
      |       if ~strcmp(fltCC1sc_bkup,tmps)
      |         set_param(gcb,'fltCC1sc',tmps);
      |       end
      |     end
      |     if isnan(fltCC2sc)
      |       if ~strcmp(fltCC2sc_bkup,'0')
      |         set_param(gcb,'fltCC2sc','0');
      |       end
      |     else
      |       tmps=num2str(fltCC2sc);
      |       if ~strcmp(fltCC2sc_bkup,tmps)
      |         set_param(gcb,'fltCC2sc',tmps);
      |       end
      |     end
      |   end
      | end
      mask TypeOptions intmethod: Forward Rectangular | Backward Rectangular | Trapezoidal
      mask Callback intmethod:
      | autoCalcEn=get_param(gcb,'autoCalcEn');
      | if strcmp(autoCalcEn,'on')
      |   SampleTime=Simulink.data.evalinGlobal(bdroot,get_param(gcb,'SampleTime'));
      |   if (SampleTime==-1)
      |     SampleTime=str2double(get_param(gcb,'SampleTime_1'));
      |   end
      |   fltCC1sc_bkup=get_param(gcb,'fltCC1sc');
      |   fltCC2sc_bkup=get_param(gcb,'fltCC2sc');
      |   intmethod=get_param(gcb,'intmethod');
      |   pgain=Simulink.data.evalinGlobal(bdroot,get_param(gcb,'pgain'));
      |   igain=Simulink.data.evalinGlobal(bdroot,get_param(gcb,'igain'));
      |   if strcmp(intmethod,'Forward Rectangular')
      |     cc1=pgain;
      |     cc2=-pgain+igain*SampleTime;
      |   else
      |     if strcmp(intmethod,'Backward Rectangular')
      |       cc1=pgain+igain*SampleTime;
      |       cc2=-pgain;
      |     else
      |       cc1=pgain+igain*SampleTime*0.5;
      |       cc2=-pgain+igain*SampleTime*0.5;
      |     end
      |   end
      |   fltCC1sc=cc1;
      |   fltCC2sc=cc2;
      |   if isnan(fltCC1sc)
      |     if ~strcmp(fltCC1sc_bkup,'0')
      |       set_param(gcb,'fltCC1sc','0');
      |     end
      |   else
      |     tmps=num2str(fltCC1sc);
      |     if ~strcmp(fltCC1sc_bkup,tmps)
      |       set_param(gcb,'fltCC1sc',tmps);
      |     end
      |   end
      |   if isnan(fltCC2sc)
      |     if ~strcmp(fltCC2sc_bkup,'0')
      |       set_param(gcb,'fltCC2sc','0');
      |     end
      |   else
      |     tmps=num2str(fltCC2sc);
      |     if ~strcmp(fltCC2sc_bkup,tmps)
      |       set_param(gcb,'fltCC2sc',tmps);
      |     end
      |   end
      | end
      mask Callback pgain:
      | autoCalcEn=get_param(gcb,'autoCalcEn');
      | if strcmp(autoCalcEn,'on')
      |   SampleTime=Simulink.data.evalinGlobal(bdroot,get_param(gcb,'SampleTime'));
      |   if (SampleTime==-1)
      |     SampleTime=str2double(get_param(gcb,'SampleTime_1'));
      |   end
      |   fltCC1sc_bkup=get_param(gcb,'fltCC1sc');
      |   fltCC2sc_bkup=get_param(gcb,'fltCC2sc');
      |   intmethod=get_param(gcb,'intmethod');
      |   pgain=Simulink.data.evalinGlobal(bdroot,get_param(gcb,'pgain'));
      |   igain=Simulink.data.evalinGlobal(bdroot,get_param(gcb,'igain'));
      |   if strcmp(intmethod,'Forward Rectangular')
      |     cc1=pgain;
      |     cc2=-pgain+igain*SampleTime;
      |   else
      |     if strcmp(intmethod,'Backward Rectangular')
      |       cc1=pgain+igain*SampleTime;
      |       cc2=-pgain;
      |     else
      |       cc1=pgain+igain*SampleTime*0.5;
      |       cc2=-pgain+igain*SampleTime*0.5;
      |     end
      |   end
      |   fltCC1sc=cc1;
      |   fltCC2sc=cc2;
      |   if isnan(fltCC1sc)
      |     if ~strcmp(fltCC1sc_bkup,'0')
      |       set_param(gcb,'fltCC1sc','0');
      |     end
      |   else
      |     tmps=num2str(fltCC1sc);
      |     if ~strcmp(fltCC1sc_bkup,tmps)
      |       set_param(gcb,'fltCC1sc',tmps);
      |     end
      |   end
      |   if isnan(fltCC2sc)
      |     if ~strcmp(fltCC2sc_bkup,'0')
      |       set_param(gcb,'fltCC2sc','0');
      |     end
      |   else
      |     tmps=num2str(fltCC2sc);
      |     if ~strcmp(fltCC2sc_bkup,tmps)
      |       set_param(gcb,'fltCC2sc',tmps);
      |     end
      |   end
      | end
      mask Callback igain:
      | autoCalcEn=get_param(gcb,'autoCalcEn');
      | if strcmp(autoCalcEn,'on')
      |   SampleTime=Simulink.data.evalinGlobal(bdroot,get_param(gcb,'SampleTime'));
      |   if (SampleTime==-1)
      |     SampleTime=str2double(get_param(gcb,'SampleTime_1'));
      |   end
      |   fltCC1sc_bkup=get_param(gcb,'fltCC1sc');
      |   fltCC2sc_bkup=get_param(gcb,'fltCC2sc');
      |   intmethod=get_param(gcb,'intmethod');
      |   pgain=Simulink.data.evalinGlobal(bdroot,get_param(gcb,'pgain'));
      |   igain=Simulink.data.evalinGlobal(bdroot,get_param(gcb,'igain'));
      |   if strcmp(intmethod,'Forward Rectangular')
      |     cc1=pgain;
      |     cc2=-pgain+igain*SampleTime;
      |   else
      |     if strcmp(intmethod,'Backward Rectangular')
      |       cc1=pgain+igain*SampleTime;
      |       cc2=-pgain;
      |     else
      |       cc1=pgain+igain*SampleTime*0.5;
      |       cc2=-pgain+igain*SampleTime*0.5;
      |     end
      |   end
      |   fltCC1sc=cc1;
      |   fltCC2sc=cc2;
      |   if isnan(fltCC1sc)
      |     if ~strcmp(fltCC1sc_bkup,'0')
      |       set_param(gcb,'fltCC1sc','0');
      |     end
      |   else
      |     tmps=num2str(fltCC1sc);
      |     if ~strcmp(fltCC1sc_bkup,tmps)
      |       set_param(gcb,'fltCC1sc',tmps);
      |     end
      |   end
      |   if isnan(fltCC2sc)
      |     if ~strcmp(fltCC2sc_bkup,'0')
      |       set_param(gcb,'fltCC2sc','0');
      |     end
      |   else
      |     tmps=num2str(fltCC2sc);
      |     if ~strcmp(fltCC2sc_bkup,tmps)
      |       set_param(gcb,'fltCC2sc',tmps);
      |     end
      |   end
      | end
      mask Callback autoCalcEn:
      | maskStr=get_param(gcb,'showStates');
      | if strcmp(maskStr,'Hide (faster execution)')
      |   p=Simulink.Mask.get(gcb);
      |   autoCalcEn=get_param(gcb,'autoCalcEn');
      |   hintText=p.getDialogControl('timeHint');
      |   if strcmp(autoCalcEn,'on')
      |     param=p.getParameter('igain');
      |     if strcmp(param.Enabled,'off')
      |       SampleTime=Simulink.data.evalinGlobal(bdroot,get_param(gcb,'SampleTime'));
      |       if SampleTime==-1
      |         SampleTime=str2double(get_param(gcb,'SampleTime_1'));
      |         if isnan(SampleTime)
      |           hintText.Prompt=['Note: Implementation parameters cannot be calculated yet because the block''s inherited sample time is unknown. Simulink will update the sample time when you run the simulation.'];
      |         else
      |           hintText.Prompt=['Caution: Implementation parameters depend on inherited sample time. Make sure that the sample time of the block''s inputs corresponds to the sampling period in the target application.'];
      |         end
      |       else
      |         hintText.Prompt='Caution: Implementation parameters depend on the sample time. Make sure that the simulation time step corresponds to the sampling period in the target application.';
      |       end
      |       p=Simulink.Mask.get(gcb);
      |       param=p.getParameter('intmethod');
      |       param.set('Enabled','on');
      |       param=p.getParameter('pgain');
      |       param.set('Enabled','on');
      |       param=p.getParameter('igain');
      |       param.set('Enabled','on');
      |     else
      |       SampleTime=Simulink.data.evalinGlobal(bdroot,get_param(gcb,'SampleTime'));
      |       if SampleTime==-1
      |         SampleTime=str2double(get_param(gcb,'SampleTime_1'));
      |       end
      |     end
      |     fltCC1sc_bkup=get_param(gcb,'fltCC1sc');
      |     fltCC2sc_bkup=get_param(gcb,'fltCC2sc');
      |     intmethod=get_param(gcb,'intmethod');
      |     pgain=Simulink.data.evalinGlobal(bdroot,get_param(gcb,'pgain'));
      |     igain=Simulink.data.evalinGlobal(bdroot,get_param(gcb,'igain'));
      |     if strcmp(intmethod,'Forward Rectangular')
      |       cc1=pgain;
      |       cc2=-pgain+igain*SampleTime;
      |     else
      |       if strcmp(intmethod,'Backward Rectangular')
      |         cc1=pgain+igain*SampleTime;
      |         cc2=-pgain;
      |       else
      |         cc1=pgain+igain*SampleTime*0.5;
      |         cc2=-pgain+igain*SampleTime*0.5;
      |       end
      |     end
      |     fltCC1sc=cc1;
      |     fltCC2sc=cc2;
      |     if isnan(fltCC1sc)
      |       if ~strcmp(fltCC1sc_bkup,'0')
      |         set_param(gcb,'fltCC1sc','0');
      |       end
      |     else
      |       tmps=num2str(fltCC1sc);
      |       if ~strcmp(fltCC1sc_bkup,tmps)
      |         set_param(gcb,'fltCC1sc',tmps);
      |       end
      |     end
      |     if isnan(fltCC2sc)
      |       if ~strcmp(fltCC2sc_bkup,'0')
      |         set_param(gcb,'fltCC2sc','0');
      |       end
      |     else
      |       tmps=num2str(fltCC2sc);
      |       if ~strcmp(fltCC2sc_bkup,tmps)
      |         set_param(gcb,'fltCC2sc',tmps);
      |       end
      |     end
      |   else
      |     param=p.getParameter('igain');
      |     if strcmp(param.Enabled,'on')
      |       hintText.Prompt='Caution: Implementation parameters are fixed.';
      |       p=Simulink.Mask.get(gcb);
      |       param=p.getParameter('intmethod');
      |       param.set('Enabled','off');
      |       param=p.getParameter('pgain');
      |       param.set('Enabled','off');
      |       param=p.getParameter('igain');
      |       param.set('Enabled','off');
      |     end
      |   end
      | end
      mask DialogControl CompBut Prompt: Recalculate sample times
      mask DialogControl CompBut Tooltip: Simulink updates the sample times of all blocks when the simulation is run. This button will update the sample times now.
      mask DialogControl CompBut Callback:
      | btn=questdlg('This will apply all changes in all open dialog boxes and update the schematic. Do you want to proceed?','Apply all changes','Continue','Cancel','Continue');
      | if strcmp(btn,'Continue')
      |   dlgs=DAStudio.ToolRoot.getOpenDialogs;
      |   for i=1:length(dlgs)
      |     dlgs(i).apply;
      |   end
      |   try
      |     SampleTime_1=str2double(get_param(gcb,'SampleTime_1'));
      |     ts=Simulink.Block.getSampleTimes(gcb);
      |     ts=ts(1).Value(1);
      |     if (SampleTime_1 ~= ts)
      |       SampleTime_1=ts;
      |       set_param(gcb,'SampleTime_1',num2str(ts));
      |       autoCalcEn=get_param(gcb,'autoCalcEn');
      |       if strcmp(autoCalcEn,'on')
      |         SampleTime=Simulink.data.evalinGlobal(bdroot,get_param(gcb,'SampleTime'));
      |         p=Simulink.Mask.get(gcb);
      |         hintText=p.getDialogControl('timeHint');
      |         if SampleTime==-1
      |           SampleTime=SampleTime_1;
      |           hintText.Prompt='Caution: Implementation parameters depend on inherited sample time. Make sure that the sample time of the block''s inputs corresponds to the sampling period in the target application.';
      |         else
      |           hintText.Prompt='Caution: Implementation parameters depend on the sample time. Make sure that the simulation time step corresponds to the sampling period in the target application.';
      |         end
      |         fltCC1sc_bkup=get_param(gcb,'fltCC1sc');
      |         fltCC2sc_bkup=get_param(gcb,'fltCC2sc');
      |         intmethod=get_param(gcb,'intmethod');
      |         pgain=Simulink.data.evalinGlobal(bdroot,get_param(gcb,'pgain'));
      |         igain=Simulink.data.evalinGlobal(bdroot,get_param(gcb,'igain'));
      |         if strcmp(intmethod,'Forward Rectangular')
      |           cc1=pgain;
      |           cc2=-pgain+igain*SampleTime;
      |         else
      |           if strcmp(intmethod,'Backward Rectangular')
      |             cc1=pgain+igain*SampleTime;
      |             cc2=-pgain;
      |           else
      |             cc1=pgain+igain*SampleTime*0.5;
      |             cc2=-pgain+igain*SampleTime*0.5;
      |           end
      |         end
      |         fltCC1sc=cc1;
      |         fltCC2sc=cc2;
      |         if isnan(fltCC1sc)
      |           if ~strcmp(fltCC1sc_bkup,'0')
      |             set_param(gcb,'fltCC1sc','0');
      |           end
      |         else
      |           tmps=num2str(fltCC1sc);
      |           if ~strcmp(fltCC1sc_bkup,tmps)
      |             set_param(gcb,'fltCC1sc',tmps);
      |           end
      |         end
      |         if isnan(fltCC2sc)
      |           if ~strcmp(fltCC2sc_bkup,'0')
      |             set_param(gcb,'fltCC2sc','0');
      |           end
      |         else
      |           tmps=num2str(fltCC2sc);
      |           if ~strcmp(fltCC2sc_bkup,tmps)
      |             set_param(gcb,'fltCC2sc',tmps);
      |           end
      |         end
      |       end
      |     end
      |   catch
      |    warning(['Sample time cannot be calculated for the block ' gcb])
      |   end
      | end
      mask DialogControl timeHint Prompt: Note: Implementation parameters cannot be calculated yet because the block's inherited sample time is unknown. Simulink will update the sample time when you run the simulation.
      mask Display:
      | color('black');
      | pos = get_param(gcb, 'Position');
      | width = pos(3) - pos(1);
      | height = pos(4) - pos(2);
      | tX=width/2;
      | tY=height - 25;
      | color('black');
      | text(tX,tY, 'GFLIB_ControllerPIr_FLT', 'horizontalAlignment', 'center');
      | if showStates == 2
      |   color('red');
      |   text(tX,tY - 20, ['debugging mode' char(13) char(10) '(limited performance)'], 'horizontalAlignment', 'center');
      | end
  GFLIB_Cos_FLT : Subsystem  TreatAsAtomicUnit=on  mask(GFLIB_Cos_FLT){}
      mask help: Cosine function in single precision floating-point implementation. Refer to the AMMCLIB User's Guide for further details.
      mask init: same as ammclib_bam_S32K3xx/GDFLIB/F16/GDFLIB_FilterFIR_F16
      settings: RTWSystemCode=Inline
      mask Help: web([fileparts(which('ammclib_bam_S32K3xx.slx')) '/../doc/S32K3XXMCLUG.pdf'], '-browser')
      mask Display: pos = get_param(gcb, 'Position');width = pos(3) - pos(1); height = pos(4) - pos(2);tX=width/2;tY=height - 8;color('black');text(tX,tY, 'GFLIB_Cos_FLT', 'horizontalAlignment', 'center');
  GFLIB_Hyst_FLT : Subsystem  TreatAsAtomicUnit=on  mask(GFLIB_Hyst_FLT){showStates=Hide (faster execution), fltHystOn=0, fltHystOff=0, fltOutValOn=0, fltOutValOff=0}
      mask prompts: showStates "Show internal states:"; fltHystOn "fltHystOn (Value determining the upper threshold):"; fltHystOff "fltHystOff (Value determining the lower threshold):"; fltOutValOn "fltOutValOn (Value of the output when input is higher than the upper threshold):"; fltOutValOff "fltOutValOff (Value of the output when input is lower than the lower threshold):"
      mask help: Hysteresis function in single precision floating-point implementation. Refer to the AMMCLIB User's Guide for further details.
      mask init:
      | ddName = get_param(bdroot,'DataDictionary');
      | if length(ddName)==0
      |   set_param(bdroot,'DataDictionary','ammclib_types.sldd');
      | else
      |   dd = Simulink.data.dictionary.open(ddName);
      |   data = getSection(dd,'Design Data');
      |   if ~exist(data,'SWLIBS_2Syst_F16')
      |     addDataSource(dd,'ammclib_types.sldd');
      |     saveChanges(dd);
      |   end
      | end
      | 
      | if showStates == 1
      |   % hidden state variables
      |   if strcmp(get_param([gcb '/fltHystOn'], 'BlockType'), 'Inport')
      |     posblk = get_param(gcb, 'Position');
      | 
      |     pos = get_param([gcb, '/fltHystOn'], 'Position');
      |     orient = get_param([gcb, '/fltHystOn'], 'Orientation');
      |     delete_block([gcb, '/fltHystOn']);
      |     add_block('built-in/Ground', [gcb, '/fltHystOn'], 'Position', pos, 'Orientation', orient);
      | 
      |     pos = get_param([gcb, '/fltHystOff'], 'Position');
      |     orient = get_param([gcb, '/fltHystOff'], 'Orientation');
      |     delete_block([gcb, '/fltHystOff']);
      |     add_block('built-in/Ground', [gcb, '/fltHystOff'], 'Position', pos, 'Orientation', orient);
      | 
      |     pos = get_param([gcb, '/fltOutValOn'], 'Position');
      |     orient = get_param([gcb, '/fltOutValOn'], 'Orientation');
      |     delete_block([gcb, '/fltOutValOn']);
      |     add_block('built-in/Ground', [gcb, '/fltOutValOn'], 'Position', pos, 'Orientation', orient);
      | 
      |     pos = get_param([gcb, '/fltOutValOff'], 'Position');
      |     orient = get_param([gcb, '/fltOutValOff'], 'Orientation');
      |     delete_block([gcb, '/fltOutValOff']);
      |     add_block('built-in/Ground', [gcb, '/fltOutValOff'], 'Position', pos, 'Orientation', orient);
      | 
      |     pos = get_param([gcb, '/fltOutState'], 'Position');
      |     orient = get_param([gcb, '/fltOutState'], 'Orientation');
      |     delete_block([gcb, '/fltOutState']);
      |     add_block('built-in/Ground', [gcb, '/fltOutState'], 'Position', pos, 'Orientation', orient);
      | 
      | 
      |     pos = get_param([gcb '/fltOutState_Out'], 'Position');
      |     orient = get_param([gcb '/fltOutState_Out'], 'Orientation');
      |     delete_block([gcb '/fltOutState_Out']);
      |     add_block('built-in/Terminator', [gcb '/fltOutState_Out'], 'Position', pos, 'Orientation', orient);
      | 
      |     set_param([gcb '/fltIn'], 'Port', '1');
      | 
      |     tmpOutCnt=0;
      |     tmpOutCnt=tmpOutCnt+1;
      |     set_param([gcb '/fltOut'], 'Port', num2str(tmpOutCnt));
      | 
      | set_param(gcb,'MaskEnables',{'on','on','on','on','on'});
      | 
      |     if (posblk(4) - posblk(2)) > 50
      |       height = 50;
      |       set_param(gcb,'Position',[posblk(1), posblk(2), posblk(3), posblk(2)+height])
      |     end
      |   end
      | else
      |   % shown state variables
      |   if strcmp(get_param([gcb '/fltHystOn'], 'BlockType'), 'Ground')
      |     posblk = get_param(gcb, 'Position');
      | 
      |     pos = get_param([gcb, '/fltHystOn'], 'Position');
      |     orient = get_param([gcb, '/fltHystOn'], 'Orientation');
      |     delete_block([gcb, '/fltHystOn']);
      |     add_block('built-in/Inport', [gcb, '/fltHystOn'], 'Position', pos, 'Orientation', orient, 'OutDataTypeStr', 'single');
      | 
      |     pos = get_param([gcb, '/fltHystOff'], 'Position');
      |     orient = get_param([gcb, '/fltHystOff'], 'Orientation');
      |     delete_block([gcb, '/fltHystOff']);
      |     add_block('built-in/Inport', [gcb, '/fltHystOff'], 'Position', pos, 'Orientation', orient, 'OutDataTypeStr', 'single');
      | 
      |     pos = get_param([gcb, '/fltOutValOn'], 'Position');
      |     orient = get_param([gcb, '/fltOutValOn'], 'Orientation');
      |     delete_block([gcb, '/fltOutValOn']);
      |     add_block('built-in/Inport', [gcb, '/fltOutValOn'], 'Position', pos, 'Orientation', orient, 'OutDataTypeStr', 'single');
      | 
      |     pos = get_param([gcb, '/fltOutValOff'], 'Position');
      |     orient = get_param([gcb, '/fltOutValOff'], 'Orientation');
      |     delete_block([gcb, '/fltOutValOff']);
      |     add_block('built-in/Inport', [gcb, '/fltOutValOff'], 'Position', pos, 'Orientation', orient, 'OutDataTypeStr', 'single');
      | 
      |     pos = get_param([gcb, '/fltOutState'], 'Position');
      |     orient = get_param([gcb, '/fltOutState'], 'Orientation');
      |     delete_block([gcb, '/fltOutState']);
      |     add_block('built-in/Inport', [gcb, '/fltOutState'], 'Position', pos, 'Orientation', orient, 'OutDataTypeStr', 'single');
      | 
      | 
      | 
      |     pos = get_param([gcb '/fltOutState_Out'], 'Position');
      |     orient = get_param([gcb '/fltOutState_Out'], 'Orientation');
      |     delete_block([gcb '/fltOutState_Out']);
      |     add_block('built-in/Outport', [gcb '/fltOutState_Out'], 'Position', pos, 'Orientation', orient);
      | 
      | 
      |     set_param([gcb '/fltIn'], 'Port', '1');
      |     set_param([gcb '/fltHystOn'], 'Port', '2');
      |     set_param([gcb '/fltHystOff'], 'Port', '3');
      |     set_param([gcb '/fltOutValOn'], 'Port', '4');
      |     set_param([gcb '/fltOutValOff'], 'Port', '5');
      |     set_param([gcb '/fltOutState'], 'Port', '6');
      | 
      |     tmpOutCnt=0;
      |     tmpOutCnt=tmpOutCnt+1;
      |     set_param([gcb '/fltOut'], 'Port', num2str(tmpOutCnt));
      |     tmpOutCnt=tmpOutCnt+1;
      |     set_param([gcb '/fltOutState_Out'], 'Port', num2str(tmpOutCnt));
      | 
      |     set_param(gcb,'MaskEnables',{'on','off','off','off','off'});
      | 
      |     if (posblk(4) - posblk(2)) < 175
      |       height = 175;
      |       set_param(gcb,'Position',[posblk(1), posblk(2), posblk(3), posblk(2)+height])
      |     end
      |   end
      | end
      settings: RTWSystemCode=Inline
      mask Help: web([fileparts(which('ammclib_bam_S32K3xx.slx')) '/../doc/S32K3XXMCLUG.pdf'], '-browser')
      mask TypeOptions showStates: Hide (faster execution) | Show (allows debugging; connect feedback loops manually)
      mask Callback showStates:
      | maskStr=get_param(gcb,'showStates');
      | if strcmp(maskStr,'Hide (faster execution)')
      |   if strcmp(get_param([gcb '/fltHystOn'], 'BlockType'), 'Inport')
      | set_param(gcb,'MaskEnables',{'on','on','on','on','on'});
      |   end
      | else
      |   if strcmp(get_param([gcb '/fltHystOn'], 'BlockType'), 'Ground')
      |     set_param(gcb,'MaskEnables',{'on','off','off','off','off'});
      |   end
      | end
      mask Display:
      | color('black');
      | pos = get_param(gcb, 'Position');
      | width = pos(3) - pos(1);
      | height = pos(4) - pos(2);
      | tX=width/2;
      | tY=height - 8;
      | color('black');
      | text(tX,tY, 'GFLIB_Hyst_FLT', 'horizontalAlignment', 'center');
      | if showStates == 2
      |   color('red');
      |   text(tX,tY - 20, ['debugging mode' char(13) char(10) '(limited performance)'], 'horizontalAlignment', 'center');
      | end
  GFLIB_IntegratorTR_FLT : Subsystem  StartFcn=|  TreatAsAtomicUnit=on  mask(GFLIB_IntegratorTR_FLT){showStates=Hide (faster execution), resetStatesEnable=Pre-set according to the first set of inputs after reset, SampleTime=-1, hiddenPlaceholder=[], autoCalcEn=on, fltC1=0, SampleTime_1=NaN}
      | ts=get_param(gcb,'CompiledSampleTime');
      | if iscell(ts)
      |   ts=ts{1};
      |   if iscell(ts)
      |     ts=ts{1};
      |   end
      | end
      | ts=ts(1);
      | set_param(gcb,'SampleTime_1',num2str(ts));
      | p=Simulink.Mask.get(gcb);
      | hintText=p.getDialogControl('timeHint');
      | SampleTime=Simulink.data.evalinGlobal(bdroot,get_param(gcb,'SampleTime'));
      | p=Simulink.Mask.get(gcb);
      | autoCalcEn=get_param(gcb,'autoCalcEn');
      | if strcmp(autoCalcEn,'on')
      |   if SampleTime==-1
      |     hintText.Prompt='Caution: Implementation parameters depend on inherited sample time. Make sure that the sample time of the block''s inputs corresponds to the sampling period in the target application.';
      |   else
      |     hintText.Prompt='Caution: Implementation parameters depend on the sample time. Make sure that the simulation time step corresponds to the sampling period in the target application.';
      |   end
      |   SampleTime=ts;
      |   fltC1_bkup=get_param(gcb,'fltC1');
      |   fltC1=SampleTime*0.5;
      |   if isnan(fltC1)
      |     if ~strcmp(fltC1_bkup,'0')
      |       set_param(gcb,'fltC1','0');
      |     end
      |   else
      |     tmps=num2str(fltC1);
      |     if ~strcmp(fltC1_bkup,tmps)
      |       set_param(gcb,'fltC1',tmps);
      |     end
      |   end
      | end
      mask prompts: showStates "Show internal states:"; resetStatesEnable "Internal state after reset:"; SampleTime "Sample time (-1 for inherited):"; autoCalcEn "Calculate implementation parameters from physical parameters"; fltC1 "fltC1 (Integrator coefficient):"; SampleTime_1 "Discrete sample time:"
      mask help: Discrete-time integrator transformed from continuous-time domain using bilinear (trapezoidal) method in single precision floating-point implementation. This block supports re-initialization of the internal state during simulation. If the block is reset, the integrator's output will be aligned with the input fltIntegratorTROut_preset. Refer to the AMMCLIB User's Guide for further details.
      mask init:
      | ddName = get_param(bdroot,'DataDictionary');
      | if length(ddName)==0
      |   set_param(bdroot,'DataDictionary','ammclib_types.sldd');
      | else
      |   dd = Simulink.data.dictionary.open(ddName);
      |   data = getSection(dd,'Design Data');
      |   if ~exist(data,'SWLIBS_2Syst_F16')
      |     addDataSource(dd,'ammclib_types.sldd');
      |     saveChanges(dd);
      |   end
      | end
      | 
      | if showStates == 1
      |   % hidden state variables
      |   if strcmp(get_param([gcb '/fltC1'], 'BlockType'), 'Inport')
      |     posblk = get_param(gcb, 'Position');
      | 
      |     pos = get_param([gcb, '/fltC1'], 'Position');
      |     orient = get_param([gcb, '/fltC1'], 'Orientation');
      |     delete_block([gcb, '/fltC1']);
      |     add_block('built-in/Ground', [gcb, '/fltC1'], 'Position', pos, 'Orientation', orient);
      | 
      |     pos = get_param([gcb, '/fltState'], 'Position');
      |     orient = get_param([gcb, '/fltState'], 'Orientation');
      |     delete_block([gcb, '/fltState']);
      |     add_block('built-in/Ground', [gcb, '/fltState'], 'Position', pos, 'Orientation', orient);
      | 
      |     pos = get_param([gcb, '/fltInK1'], 'Position');
      |     orient = get_param([gcb, '/fltInK1'], 'Orientation');
      |     delete_block([gcb, '/fltInK1']);
      |     add_block('built-in/Ground', [gcb, '/fltInK1'], 'Position', pos, 'Orientation', orient);
      | 
      | 
      |     pmask=Simulink.Mask.get(gcb);
      |     pctrl=pmask.getParameter('SampleTime');
      |     pctrl.set('TypeOptions',{'fltIn/SampleTime','fltIntegratorTROut_preset/SampleTime'});
      | 
      |     pos = get_param([gcb '/fltState_Out'], 'Position');
      |     orient = get_param([gcb '/fltState_Out'], 'Orientation');
      |     delete_block([gcb '/fltState_Out']);
      |     add_block('built-in/Terminator', [gcb '/fltState_Out'], 'Position', pos, 'Orientation', orient);
      | 
      |     pos = get_param([gcb '/fltInK1_Out'], 'Position');
      |     orient = get_param([gcb '/fltInK1_Out'], 'Orientation');
      |     delete_block([gcb '/fltInK1_Out']);
      |     add_block('built-in/Terminator', [gcb '/fltInK1_Out'], 'Position', pos, 'Orientation', orient);
      | 
      |     set_param([gcb '/fltIn'], 'Port', '1');
      |     set_param([gcb '/fltIntegratorTROut_preset'], 'Port', '2');
      | 
      |     tmpOutCnt=0;
      |     tmpOutCnt=tmpOutCnt+1;
      |     set_param([gcb '/fltOut'], 'Port', num2str(tmpOutCnt));
      | 
      |     autoCalcEn=get_param(gcb,'autoCalcEn');
      |     if strcmp(autoCalcEn,'on')
      |       set_param(gcb,'MaskEnables',{'on','on','on','on','on','on','off'});
      |     else
      |       set_param(gcb,'MaskEnables',{'on','on','on','off','on','on','off'});
      |     end
      | 
      |     if (posblk(4) - posblk(2)) > 75
      |       height = 75;
      |       set_param(gcb,'Position',[posblk(1), posblk(2), posblk(3), posblk(2)+height])
      |     end
      |   end
      | else
      |   % shown state variables
      |   if strcmp(get_param([gcb '/fltC1'], 'BlockType'), 'Ground')
      |     posblk = get_param(gcb, 'Position');
      | 
      |     pos = get_param([gcb, '/fltC1'], 'Position');
      |     orient = get_param([gcb, '/fltC1'], 'Orientation');
      |     delete_block([gcb, '/fltC1']);
      |     add_block('built-in/Inport', [gcb, '/fltC1'], 'Position', pos, 'Orientation', orient, 'OutDataTypeStr', 'single');
      | 
      |     pos = get_param([gcb, '/fltState'], 'Position');
      |     orient = get_param([gcb, '/fltState'], 'Orientation');
      |     delete_block([gcb, '/fltState']);
      |     add_block('built-in/Inport', [gcb, '/fltState'], 'Position', pos, 'Orientation', orient, 'OutDataTypeStr', 'single');
      | 
      |     pos = get_param([gcb, '/fltInK1'], 'Position');
      |     orient = get_param([gcb, '/fltInK1'], 'Orientation');
      |     delete_block([gcb, '/fltInK1']);
      |     add_block('built-in/Inport', [gcb, '/fltInK1'], 'Position', pos, 'Orientation', orient, 'OutDataTypeStr', 'single');
      | 
      | 
      | 
      |     pos = get_param([gcb '/fltState_Out'], 'Position');
      |     orient = get_param([gcb '/fltState_Out'], 'Orientation');
      |     delete_block([gcb '/fltState_Out']);
      |     add_block('built-in/Outport', [gcb '/fltState_Out'], 'Position', pos, 'Orientation', orient);
      | 
      |     pos = get_param([gcb '/fltInK1_Out'], 'Position');
      |     orient = get_param([gcb '/fltInK1_Out'], 'Orientation');
      |     delete_block([gcb '/fltInK1_Out']);
      |     add_block('built-in/Outport', [gcb '/fltInK1_Out'], 'Position', pos, 'Orientation', orient);
      | 
      | 
      |     pmask=Simulink.Mask.get(gcb);
      |     pctrl=pmask.getParameter('SampleTime');
      |     pctrl.set('TypeOptions',{'fltIn/SampleTime','fltIntegratorTROut_preset/SampleTime','fltC1/SampleTime','fltState/SampleTime','fltInK1/SampleTime'});
      | 
      |     set_param([gcb '/fltIn'], 'Port', '1');
      |     set_param([gcb '/fltIntegratorTROut_preset'], 'Port', '2');
      |     set_param([gcb '/fltC1'], 'Port', '3');
      |     set_param([gcb '/fltState'], 'Port', '4');
      |     set_param([gcb '/fltInK1'], 'Port', '5');
      | 
      |     tmpOutCnt=0;
      |     tmpOutCnt=tmpOutCnt+1;
      |     set_param([gcb '/fltOut'], 'Port', num2str(tmpOutCnt));
      |     tmpOutCnt=tmpOutCnt+1;
      |     set_param([gcb '/fltState_Out'], 'Port', num2str(tmpOutCnt));
      |     tmpOutCnt=tmpOutCnt+1;
      |     set_param([gcb '/fltInK1_Out'], 'Port', num2str(tmpOutCnt));
      | 
      |     set_param(gcb,'MaskEnables',{'on','on','on','off','off','off','off'});
      | 
      |     if (posblk(4) - posblk(2)) < 150
      |       height = 150;
      |       set_param(gcb,'Position',[posblk(1), posblk(2), posblk(3), posblk(2)+height])
      |     end
      |   end
      | end
      settings: RTWSystemCode=Inline
      mask Help: web([fileparts(which('ammclib_bam_S32K3xx.slx')) '/../doc/S32K3XXMCLUG.pdf'], '-browser')
      mask TypeOptions showStates: Hide (faster execution) | Show (allows debugging; connect feedback loops manually)
      mask Callback showStates:
      | maskStr=get_param(gcb,'showStates');
      | if strcmp(maskStr,'Hide (faster execution)')
      |   if strcmp(get_param([gcb '/fltC1'], 'BlockType'), 'Inport')
      |     autoCalcEn=get_param(gcb,'autoCalcEn');
      |     if strcmp(autoCalcEn,'on')
      |       set_param(gcb,'MaskEnables',{'on','on','on','on','on','on','off'});
      |     else
      |       set_param(gcb,'MaskEnables',{'on','on','on','off','on','on','off'});
      |     end
      |   end
      | else
      |   if strcmp(get_param([gcb '/fltC1'], 'BlockType'), 'Ground')
      |     set_param(gcb,'MaskEnables',{'on','on','on','off','off','off','off'});
      |   end
      | end
      mask TypeOptions resetStatesEnable: Pre-set according to the first set of inputs after reset | Clear to zero
      mask TypeOptions SampleTime: fltIn/SampleTime | fltIntegratorTROut_preset/SampleTime
      mask Callback SampleTime:
      | p=Simulink.Mask.get(gcb);
      | hintText=p.getDialogControl('timeHint');
      | SampleTime=Simulink.data.evalinGlobal(bdroot,get_param(gcb,'SampleTime'));
      | SampleTime_1=str2double(get_param(gcb,'SampleTime_1'));
      | if (((SampleTime==-1) && (~contains(hintText.Prompt,'inherited'))) || ...
      |     ((SampleTime~=-1) && contains(hintText.Prompt,'inherited')) || ...
      |     ((SampleTime~=-1) && (SampleTime_1~=SampleTime)) || ...
      |     ((SampleTime_1~=-1) && contains(hintText.Prompt,'yet')))
      |   if ((SampleTime==-1) && (~contains(hintText.Prompt,'inherited')))
      |     set_param(gcb,'SampleTime_1',num2str(NaN));
      |     SampleTime_1=NaN;
      |   end
      |   if (SampleTime~=-1)
      |     set_param(gcb,'SampleTime_1',num2str(SampleTime));
      |     SampleTime_1=SampleTime;
      |   end
      |   autoCalcEn=get_param(gcb,'autoCalcEn');
      |   if strcmp(autoCalcEn,'on')
      |     p=Simulink.Mask.get(gcb);
      |     hintText=p.getDialogControl('timeHint');
      |     if SampleTime==-1
      |       SampleTime=SampleTime_1;
      |       if isnan(SampleTime)
      |         hintText.Prompt='Note: Implementation parameters cannot be calculated yet because the block''s inherited sample time is unknown. Simulink will update the sample time when you run the simulation.';
      |       else
      |         hintText.Prompt='Caution: Implementation parameters depend on inherited sample time. Make sure that the sample time of the block''s inputs corresponds to the sampling period in the target application.';
      |       end
      |     else
      |       hintText.Prompt='Caution: Implementation parameters depend on the sample time. Make sure that the simulation time step corresponds to the sampling period in the target application.';
      |     end
      |     fltC1_bkup=get_param(gcb,'fltC1');
      |     fltC1=SampleTime*0.5;
      |     if isnan(fltC1)
      |       if ~strcmp(fltC1_bkup,'0')
      |         set_param(gcb,'fltC1','0');
      |       end
      |     else
      |       tmps=num2str(fltC1);
      |       if ~strcmp(fltC1_bkup,tmps)
      |         set_param(gcb,'fltC1',tmps);
      |       end
      |     end
      |   end
      | end
      mask Callback autoCalcEn:
      | maskStr=get_param(gcb,'showStates');
      | if strcmp(maskStr,'Hide (faster execution)')
      |   p=Simulink.Mask.get(gcb);
      |   autoCalcEn=get_param(gcb,'autoCalcEn');
      |   hintText=p.getDialogControl('timeHint');
      |   if strcmp(autoCalcEn,'on')
      |     param=p.getParameter('hiddenPlaceholder');
      |     if strcmp(param.Enabled,'off')
      |       SampleTime=Simulink.data.evalinGlobal(bdroot,get_param(gcb,'SampleTime'));
      |       if SampleTime==-1
      |         SampleTime=str2double(get_param(gcb,'SampleTime_1'));
      |         if isnan(SampleTime)
      |           hintText.Prompt=['Note: Implementation parameters cannot be calculated yet because the block''s inherited sample time is unknown. Simulink will update the sample time when you run the simulation.'];
      |         else
      |           hintText.Prompt=['Caution: Implementation parameters depend on inherited sample time. Make sure that the sample time of the block''s inputs corresponds to the sampling period in the target application.'];
      |         end
      |       else
      |         hintText.Prompt='Caution: Implementation parameters depend on the sample time. Make sure that the simulation time step corresponds to the sampling period in the target application.';
      |       end
      |       p=Simulink.Mask.get(gcb);
      |       param=p.getParameter('hiddenPlaceholder');
      |       param.set('Enabled','on');
      |     else
      |       SampleTime=Simulink.data.evalinGlobal(bdroot,get_param(gcb,'SampleTime'));
      |       if SampleTime==-1
      |         SampleTime=str2double(get_param(gcb,'SampleTime_1'));
      |       end
      |     end
      |     fltC1_bkup=get_param(gcb,'fltC1');
      |     hiddenPlaceholder=Simulink.data.evalinGlobal(bdroot,get_param(gcb,'hiddenPlaceholder'));
      |     fltC1=SampleTime*0.5;
      |     if isnan(fltC1)
      |       if ~strcmp(fltC1_bkup,'0')
      |         set_param(gcb,'fltC1','0');
      |       end
      |     else
      |       tmps=num2str(fltC1);
      |       if ~strcmp(fltC1_bkup,tmps)
      |         set_param(gcb,'fltC1',tmps);
      |       end
      |     end
      |   else
      |     param=p.getParameter('hiddenPlaceholder');
      |     if strcmp(param.Enabled,'on')
      |       hintText.Prompt='Caution: Implementation parameters are fixed.';
      |       p=Simulink.Mask.get(gcb);
      |       param=p.getParameter('hiddenPlaceholder');
      |       param.set('Enabled','off');
      |     end
      |   end
      | end
      mask DialogControl nophyText Prompt: No manually edited continuous-time parameters.
      mask DialogControl CompBut Prompt: Recalculate sample times
      mask DialogControl CompBut Tooltip: Simulink updates the sample times of all blocks when the simulation is run. This button will update the sample times now.
      mask DialogControl CompBut Callback:
      | btn=questdlg('This will apply all changes in all open dialog boxes and update the schematic. Do you want to proceed?','Apply all changes','Continue','Cancel','Continue');
      | if strcmp(btn,'Continue')
      |   dlgs=DAStudio.ToolRoot.getOpenDialogs;
      |   for i=1:length(dlgs)
      |     dlgs(i).apply;
      |   end
      |   try
      |     SampleTime_1=str2double(get_param(gcb,'SampleTime_1'));
      |     ts=Simulink.Block.getSampleTimes(gcb);
      |     ts=ts(1).Value(1);
      |     if (SampleTime_1 ~= ts)
      |       SampleTime_1=ts;
      |       set_param(gcb,'SampleTime_1',num2str(ts));
      |       autoCalcEn=get_param(gcb,'autoCalcEn');
      |       if strcmp(autoCalcEn,'on')
      |         SampleTime=Simulink.data.evalinGlobal(bdroot,get_param(gcb,'SampleTime'));
      |         p=Simulink.Mask.get(gcb);
      |         hintText=p.getDialogControl('timeHint');
      |         if SampleTime==-1
      |           SampleTime=SampleTime_1;
      |           hintText.Prompt='Caution: Implementation parameters depend on inherited sample time. Make sure that the sample time of the block''s inputs corresponds to the sampling period in the target application.';
      |         else
      |           hintText.Prompt='Caution: Implementation parameters depend on the sample time. Make sure that the simulation time step corresponds to the sampling period in the target application.';
      |         end
      |         fltC1_bkup=get_param(gcb,'fltC1');
      |         hiddenPlaceholder=Simulink.data.evalinGlobal(bdroot,get_param(gcb,'hiddenPlaceholder'));
      |         fltC1=SampleTime*0.5;
      |         if isnan(fltC1)
      |           if ~strcmp(fltC1_bkup,'0')
      |             set_param(gcb,'fltC1','0');
      |           end
      |         else
      |           tmps=num2str(fltC1);
      |           if ~strcmp(fltC1_bkup,tmps)
      |             set_param(gcb,'fltC1',tmps);
      |           end
      |         end
      |       end
      |     end
      |   catch
      |    warning(['Sample time cannot be calculated for the block ' gcb])
      |   end
      | end
      mask DialogControl timeHint Prompt: Note: Implementation parameters cannot be calculated yet because the block's inherited sample time is unknown. Simulink will update the sample time when you run the simulation.
      mask Display:
      | color('black');
      | pos = get_param(gcb, 'Position');
      | width = pos(3) - pos(1);
      | height = pos(4) - pos(2);
      | tX=width/2;
      | tY=height - 25;
      | color('black');
      | text(tX,tY, 'GFLIB_IntegratorTR_FLT', 'horizontalAlignment', 'center');
      | if showStates == 2
      |   color('red');
      |   text(tX,tY - 20, ['debugging mode' char(13) char(10) '(limited performance)'], 'horizontalAlignment', 'center');
      | end
  GFLIB_Limit_FLT : Subsystem  TreatAsAtomicUnit=on  mask(GFLIB_Limit_FLT){showStates=Hide (faster execution), fltLowerLimit=0, fltUpperLimit=0}
      mask prompts: showStates "Show parameters as inputs:"; fltLowerLimit "fltLowerLimit (Lower limit):"; fltUpperLimit "fltUpperLimit (Upper limit):"
      mask help: Limit function in single precision floating-point implementation. Refer to the AMMCLIB User's Guide for further details.
      mask init:
      | ddName = get_param(bdroot,'DataDictionary');
      | if length(ddName)==0
      |   set_param(bdroot,'DataDictionary','ammclib_types.sldd');
      | else
      |   dd = Simulink.data.dictionary.open(ddName);
      |   data = getSection(dd,'Design Data');
      |   if ~exist(data,'SWLIBS_2Syst_F16')
      |     addDataSource(dd,'ammclib_types.sldd');
      |     saveChanges(dd);
      |   end
      | end
      | 
      | if showStates == 1
      |   % hidden state variables
      |   if strcmp(get_param([gcb '/fltLowerLimit'], 'BlockType'), 'Inport')
      |     posblk = get_param(gcb, 'Position');
      | 
      |     pos = get_param([gcb, '/fltLowerLimit'], 'Position');
      |     orient = get_param([gcb, '/fltLowerLimit'], 'Orientation');
      |     delete_block([gcb, '/fltLowerLimit']);
      |     add_block('built-in/Ground', [gcb, '/fltLowerLimit'], 'Position', pos, 'Orientation', orient);
      | 
      |     pos = get_param([gcb, '/fltUpperLimit'], 'Position');
      |     orient = get_param([gcb, '/fltUpperLimit'], 'Orientation');
      |     delete_block([gcb, '/fltUpperLimit']);
      |     add_block('built-in/Ground', [gcb, '/fltUpperLimit'], 'Position', pos, 'Orientation', orient);
      | 
      | 
      |     set_param([gcb '/fltIn'], 'Port', '1');
      | 
      |     tmpOutCnt=0;
      |     tmpOutCnt=tmpOutCnt+1;
      |     set_param([gcb '/fltOut'], 'Port', num2str(tmpOutCnt));
      | 
      | set_param(gcb,'MaskEnables',{'on','on','on'});
      | 
      |     if (posblk(4) - posblk(2)) > 50
      |       height = 50;
      |       set_param(gcb,'Position',[posblk(1), posblk(2), posblk(3), posblk(2)+height])
      |     end
      |   end
      | else
      |   % shown state variables
      |   if strcmp(get_param([gcb '/fltLowerLimit'], 'BlockType'), 'Ground')
      |     posblk = get_param(gcb, 'Position');
      | 
      |     pos = get_param([gcb, '/fltLowerLimit'], 'Position');
      |     orient = get_param([gcb, '/fltLowerLimit'], 'Orientation');
      |     delete_block([gcb, '/fltLowerLimit']);
      |     add_block('built-in/Inport', [gcb, '/fltLowerLimit'], 'Position', pos, 'Orientation', orient, 'OutDataTypeStr', 'single');
      | 
      |     pos = get_param([gcb, '/fltUpperLimit'], 'Position');
      |     orient = get_param([gcb, '/fltUpperLimit'], 'Orientation');
      |     delete_block([gcb, '/fltUpperLimit']);
      |     add_block('built-in/Inport', [gcb, '/fltUpperLimit'], 'Position', pos, 'Orientation', orient, 'OutDataTypeStr', 'single');
      | 
      | 
      | 
      | 
      |     set_param([gcb '/fltIn'], 'Port', '1');
      |     set_param([gcb '/fltLowerLimit'], 'Port', '2');
      |     set_param([gcb '/fltUpperLimit'], 'Port', '3');
      | 
      |     tmpOutCnt=0;
      |     tmpOutCnt=tmpOutCnt+1;
      |     set_param([gcb '/fltOut'], 'Port', num2str(tmpOutCnt));
      | 
      |     set_param(gcb,'MaskEnables',{'on','off','off'});
      | 
      |     if (posblk(4) - posblk(2)) < 100
      |       height = 100;
      |       set_param(gcb,'Position',[posblk(1), posblk(2), posblk(3), posblk(2)+height])
      |     end
      |   end
      | end
      settings: RTWSystemCode=Inline
      mask Help: web([fileparts(which('ammclib_bam_S32K3xx.slx')) '/../doc/S32K3XXMCLUG.pdf'], '-browser')
      mask TypeOptions showStates: Hide (faster execution) | Show (parameters can be changed during simulation)
      mask Callback showStates:
      | maskStr=get_param(gcb,'showStates');
      | if strcmp(maskStr,'Hide (faster execution)')
      |   if strcmp(get_param([gcb '/fltLowerLimit'], 'BlockType'), 'Inport')
      | set_param(gcb,'MaskEnables',{'on','on','on'});
      |   end
      | else
      |   if strcmp(get_param([gcb '/fltLowerLimit'], 'BlockType'), 'Ground')
      |     set_param(gcb,'MaskEnables',{'on','off','off'});
      |   end
      | end
      mask Display:
      | color('black');
      | pos = get_param(gcb, 'Position');
      | width = pos(3) - pos(1);
      | height = pos(4) - pos(2);
      | tX=width/2;
      | tY=height - 8;
      | color('black');
      | text(tX,tY, 'GFLIB_Limit_FLT', 'horizontalAlignment', 'center');
      | if showStates == 2
      |   color('red');
      |   text(tX,tY - 20, ['debugging mode' char(13) char(10) '(limited performance)'], 'horizontalAlignment', 'center');
      | end
  GFLIB_Log10_FLT : Subsystem  TreatAsAtomicUnit=on  mask(GFLIB_Log10_FLT){}
      mask help: Fast base-10 logarithm function in single precision floating-point implementation. Refer to the AMMCLIB User's Guide for further details.
      mask init: same as ammclib_bam_S32K3xx/GDFLIB/F16/GDFLIB_FilterFIR_F16
      settings: RTWSystemCode=Inline
      mask Help: web([fileparts(which('ammclib_bam_S32K3xx.slx')) '/../doc/S32K3XXMCLUG.pdf'], '-browser')
      mask Display: pos = get_param(gcb, 'Position');width = pos(3) - pos(1); height = pos(4) - pos(2);tX=width/2;tY=height - 8;color('black');text(tX,tY, 'GFLIB_Log10_FLT', 'horizontalAlignment', 'center');
  GFLIB_LowerLimit_FLT : Subsystem  TreatAsAtomicUnit=on  mask(GFLIB_LowerLimit_FLT){showStates=Hide (faster execution), fltLowerLimit=0}
      mask prompts: showStates "Show parameters as inputs:"; fltLowerLimit "fltLowerLimit (Value determining the lower limit threshold):"
      mask help: Lower limit function in single precision floating-point implementation. Refer to the AMMCLIB User's Guide for further details.
      mask init:
      | ddName = get_param(bdroot,'DataDictionary');
      | if length(ddName)==0
      |   set_param(bdroot,'DataDictionary','ammclib_types.sldd');
      | else
      |   dd = Simulink.data.dictionary.open(ddName);
      |   data = getSection(dd,'Design Data');
      |   if ~exist(data,'SWLIBS_2Syst_F16')
      |     addDataSource(dd,'ammclib_types.sldd');
      |     saveChanges(dd);
      |   end
      | end
      | 
      | if showStates == 1
      |   % hidden state variables
      |   if strcmp(get_param([gcb '/fltLowerLimit'], 'BlockType'), 'Inport')
      |     posblk = get_param(gcb, 'Position');
      | 
      |     pos = get_param([gcb, '/fltLowerLimit'], 'Position');
      |     orient = get_param([gcb, '/fltLowerLimit'], 'Orientation');
      |     delete_block([gcb, '/fltLowerLimit']);
      |     add_block('built-in/Ground', [gcb, '/fltLowerLimit'], 'Position', pos, 'Orientation', orient);
      | 
      | 
      |     set_param([gcb '/fltIn'], 'Port', '1');
      | 
      |     tmpOutCnt=0;
      |     tmpOutCnt=tmpOutCnt+1;
      |     set_param([gcb '/fltOut'], 'Port', num2str(tmpOutCnt));
      | 
      | set_param(gcb,'MaskEnables',{'on','on'});
      | 
      |     if (posblk(4) - posblk(2)) > 50
      |       height = 50;
      |       set_param(gcb,'Position',[posblk(1), posblk(2), posblk(3), posblk(2)+height])
      |     end
      |   end
      | else
      |   % shown state variables
      |   if strcmp(get_param([gcb '/fltLowerLimit'], 'BlockType'), 'Ground')
      |     posblk = get_param(gcb, 'Position');
      | 
      |     pos = get_param([gcb, '/fltLowerLimit'], 'Position');
      |     orient = get_param([gcb, '/fltLowerLimit'], 'Orientation');
      |     delete_block([gcb, '/fltLowerLimit']);
      |     add_block('built-in/Inport', [gcb, '/fltLowerLimit'], 'Position', pos, 'Orientation', orient, 'OutDataTypeStr', 'single');
      | 
      | 
      | 
      | 
      |     set_param([gcb '/fltIn'], 'Port', '1');
      |     set_param([gcb '/fltLowerLimit'], 'Port', '2');
      | 
      |     tmpOutCnt=0;
      |     tmpOutCnt=tmpOutCnt+1;
      |     set_param([gcb '/fltOut'], 'Port', num2str(tmpOutCnt));
      | 
      |     set_param(gcb,'MaskEnables',{'on','off'});
      | 
      |     if (posblk(4) - posblk(2)) < 75
      |       height = 75;
      |       set_param(gcb,'Position',[posblk(1), posblk(2), posblk(3), posblk(2)+height])
      |     end
      |   end
      | end
      settings: RTWSystemCode=Inline
      mask Help: web([fileparts(which('ammclib_bam_S32K3xx.slx')) '/../doc/S32K3XXMCLUG.pdf'], '-browser')
      mask TypeOptions showStates: Hide (faster execution) | Show (parameters can be changed during simulation)
      mask Callback showStates:
      | maskStr=get_param(gcb,'showStates');
      | if strcmp(maskStr,'Hide (faster execution)')
      |   if strcmp(get_param([gcb '/fltLowerLimit'], 'BlockType'), 'Inport')
      | set_param(gcb,'MaskEnables',{'on','on'});
      |   end
      | else
      |   if strcmp(get_param([gcb '/fltLowerLimit'], 'BlockType'), 'Ground')
      |     set_param(gcb,'MaskEnables',{'on','off'});
      |   end
      | end
      mask Display:
      | color('black');
      | pos = get_param(gcb, 'Position');
      | width = pos(3) - pos(1);
      | height = pos(4) - pos(2);
      | tX=width/2;
      | tY=height - 8;
      | color('black');
      | text(tX,tY, 'GFLIB_LowerLimit_FLT', 'horizontalAlignment', 'center');
      | if showStates == 2
      |   color('red');
      |   text(tX,tY - 20, ['debugging mode' char(13) char(10) '(limited performance)'], 'horizontalAlignment', 'center');
      | end
  GFLIB_Lut1D_FLT : Subsystem  TreatAsAtomicUnit=on  mask(GFLIB_Lut1D_FLT){pfltTable=[-0.75 -0.25 0.0 0.25 0.75], s32MidIdx=2}
      mask prompts: pfltTable "pfltTable (Vector holding the ordinate values of interpolating intervals):"; s32MidIdx "Middle index in the table (zero-based indexing). This index is added to pfltTable to allow shifting the origin of the table to any point within the table:"
      mask help: One dimensional lookup table function in single precision floating-point implementation. Refer to the AMMCLIB User's Guide for further details.
      mask init: same as ammclib_bam_S32K3xx/GDFLIB/F16/GDFLIB_FilterFIR_F16
      settings: RTWSystemCode=Inline
      mask Help: web([fileparts(which('ammclib_bam_S32K3xx.slx')) '/../doc/S32K3XXMCLUG.pdf'], '-browser')
      mask Display: pos = get_param(gcb, 'Position');width = pos(3) - pos(1); height = pos(4) - pos(2);tX=width/2;tY=height - 8;color('black');text(tX,tY, 'GFLIB_Lut1D_FLT', 'horizontalAlignment', 'center');
  GFLIB_Lut2D_FLT : Subsystem  TreatAsAtomicUnit=on  mask(GFLIB_Lut2D_FLT){pfltTable=[-0.75 0.0 0.75; -0.5 0.0 0.5; -0.25 0.0 0.25], s32MidIdx=4}
      mask prompts: pfltTable "pfltTable (Matrix of z-coordinate values at vertices):"; s32MidIdx "Middle index in the table (zero-based indexing over all elements). This index is added to pfltTable to allow shifting the origin of the table coordinates to any point within the table:"
      mask help: Two dimensional lookup table function in single precision floating-point implementation. Refer to the AMMCLIB User's Guide for further details.
      mask init: same as ammclib_bam_S32K3xx/GDFLIB/F16/GDFLIB_FilterFIR_F16
      settings: RTWSystemCode=Inline
      mask Help: web([fileparts(which('ammclib_bam_S32K3xx.slx')) '/../doc/S32K3XXMCLUG.pdf'], '-browser')
      mask Display: pos = get_param(gcb, 'Position');width = pos(3) - pos(1); height = pos(4) - pos(2);tX=width/2;tY=height - 8;color('black');text(tX,tY, 'GFLIB_Lut2D_FLT', 'horizontalAlignment', 'center');
  GFLIB_Ramp_FLT : Subsystem  TreatAsAtomicUnit=on  mask(GFLIB_Ramp_FLT){showStates=Hide (faster execution), fltRampUp=0, fltRampDown=0}
      mask prompts: showStates "Show internal states:"; fltRampUp "fltRampUp (Ramp up increment coefficient):"; fltRampDown "fltRampDown (Ramp decrement coefficient):"
      mask help: Rate of change limiter - ramp function in single precision floating-point implementation. Refer to the AMMCLIB User's Guide for further details.
      mask init:
      | ddName = get_param(bdroot,'DataDictionary');
      | if length(ddName)==0
      |   set_param(bdroot,'DataDictionary','ammclib_types.sldd');
      | else
      |   dd = Simulink.data.dictionary.open(ddName);
      |   data = getSection(dd,'Design Data');
      |   if ~exist(data,'SWLIBS_2Syst_F16')
      |     addDataSource(dd,'ammclib_types.sldd');
      |     saveChanges(dd);
      |   end
      | end
      | 
      | if showStates == 1
      |   % hidden state variables
      |   if strcmp(get_param([gcb '/fltState'], 'BlockType'), 'Inport')
      |     posblk = get_param(gcb, 'Position');
      | 
      |     pos = get_param([gcb, '/fltState'], 'Position');
      |     orient = get_param([gcb, '/fltState'], 'Orientation');
      |     delete_block([gcb, '/fltState']);
      |     add_block('built-in/Ground', [gcb, '/fltState'], 'Position', pos, 'Orientation', orient);
      | 
      |     pos = get_param([gcb, '/fltRampUp'], 'Position');
      |     orient = get_param([gcb, '/fltRampUp'], 'Orientation');
      |     delete_block([gcb, '/fltRampUp']);
      |     add_block('built-in/Ground', [gcb, '/fltRampUp'], 'Position', pos, 'Orientation', orient);
      | 
      |     pos = get_param([gcb, '/fltRampDown'], 'Position');
      |     orient = get_param([gcb, '/fltRampDown'], 'Orientation');
      |     delete_block([gcb, '/fltRampDown']);
      |     add_block('built-in/Ground', [gcb, '/fltRampDown'], 'Position', pos, 'Orientation', orient);
      | 
      | 
      |     pos = get_param([gcb '/fltState_Out'], 'Position');
      |     orient = get_param([gcb '/fltState_Out'], 'Orientation');
      |     delete_block([gcb '/fltState_Out']);
      |     add_block('built-in/Terminator', [gcb '/fltState_Out'], 'Position', pos, 'Orientation', orient);
      | 
      |     set_param([gcb '/fltIn'], 'Port', '1');
      | 
      |     tmpOutCnt=0;
      |     tmpOutCnt=tmpOutCnt+1;
      |     set_param([gcb '/fltOut'], 'Port', num2str(tmpOutCnt));
      | 
      | set_param(gcb,'MaskEnables',{'on','on','on'});
      | 
      |     if (posblk(4) - posblk(2)) > 50
      |       height = 50;
      |       set_param(gcb,'Position',[posblk(1), posblk(2), posblk(3), posblk(2)+height])
      |     end
      |   end
      | else
      |   % shown state variables
      |   if strcmp(get_param([gcb '/fltState'], 'BlockType'), 'Ground')
      |     posblk = get_param(gcb, 'Position');
      | 
      |     pos = get_param([gcb, '/fltState'], 'Position');
      |     orient = get_param([gcb, '/fltState'], 'Orientation');
      |     delete_block([gcb, '/fltState']);
      |     add_block('built-in/Inport', [gcb, '/fltState'], 'Position', pos, 'Orientation', orient, 'OutDataTypeStr', 'single');
      | 
      |     pos = get_param([gcb, '/fltRampUp'], 'Position');
      |     orient = get_param([gcb, '/fltRampUp'], 'Orientation');
      |     delete_block([gcb, '/fltRampUp']);
      |     add_block('built-in/Inport', [gcb, '/fltRampUp'], 'Position', pos, 'Orientation', orient, 'OutDataTypeStr', 'single');
      | 
      |     pos = get_param([gcb, '/fltRampDown'], 'Position');
      |     orient = get_param([gcb, '/fltRampDown'], 'Orientation');
      |     delete_block([gcb, '/fltRampDown']);
      |     add_block('built-in/Inport', [gcb, '/fltRampDown'], 'Position', pos, 'Orientation', orient, 'OutDataTypeStr', 'single');
      | 
      | 
      | 
      |     pos = get_param([gcb '/fltState_Out'], 'Position');
      |     orient = get_param([gcb '/fltState_Out'], 'Orientation');
      |     delete_block([gcb '/fltState_Out']);
      |     add_block('built-in/Outport', [gcb '/fltState_Out'], 'Position', pos, 'Orientation', orient);
      | 
      | 
      |     set_param([gcb '/fltIn'], 'Port', '1');
      |     set_param([gcb '/fltState'], 'Port', '2');
      |     set_param([gcb '/fltRampUp'], 'Port', '3');
      |     set_param([gcb '/fltRampDown'], 'Port', '4');
      | 
      |     tmpOutCnt=0;
      |     tmpOutCnt=tmpOutCnt+1;
      |     set_param([gcb '/fltOut'], 'Port', num2str(tmpOutCnt));
      |     tmpOutCnt=tmpOutCnt+1;
      |     set_param([gcb '/fltState_Out'], 'Port', num2str(tmpOutCnt));
      | 
      |     set_param(gcb,'MaskEnables',{'on','off','off'});
      | 
      |     if (posblk(4) - posblk(2)) < 125
      |       height = 125;
      |       set_param(gcb,'Position',[posblk(1), posblk(2), posblk(3), posblk(2)+height])
      |     end
      |   end
      | end
      settings: RTWSystemCode=Inline
      mask Help: web([fileparts(which('ammclib_bam_S32K3xx.slx')) '/../doc/S32K3XXMCLUG.pdf'], '-browser')
      mask TypeOptions showStates: Hide (faster execution) | Show (allows debugging; connect feedback loops manually)
      mask Callback showStates:
      | maskStr=get_param(gcb,'showStates');
      | if strcmp(maskStr,'Hide (faster execution)')
      |   if strcmp(get_param([gcb '/fltState'], 'BlockType'), 'Inport')
      | set_param(gcb,'MaskEnables',{'on','on','on'});
      |   end
      | else
      |   if strcmp(get_param([gcb '/fltState'], 'BlockType'), 'Ground')
      |     set_param(gcb,'MaskEnables',{'on','off','off'});
      |   end
      | end
      mask Display:
      | color('black');
      | pos = get_param(gcb, 'Position');
      | width = pos(3) - pos(1);
      | height = pos(4) - pos(2);
      | tX=width/2;
      | tY=height - 8;
      | color('black');
      | text(tX,tY, 'GFLIB_Ramp_FLT', 'horizontalAlignment', 'center');
      | if showStates == 2
      |   color('red');
      |   text(tX,tY - 20, ['debugging mode' char(13) char(10) '(limited performance)'], 'horizontalAlignment', 'center');
      | end
  GFLIB_Sign_FLT : Subsystem  TreatAsAtomicUnit=on  mask(GFLIB_Sign_FLT){}
      mask help: Sign function in single precision floating-point implementation. Refer to the AMMCLIB User's Guide for further details.
      mask init: same as ammclib_bam_S32K3xx/GDFLIB/F16/GDFLIB_FilterFIR_F16
      settings: RTWSystemCode=Inline
      mask Help: web([fileparts(which('ammclib_bam_S32K3xx.slx')) '/../doc/S32K3XXMCLUG.pdf'], '-browser')
      mask Display: pos = get_param(gcb, 'Position');width = pos(3) - pos(1); height = pos(4) - pos(2);tX=width/2;tY=height - 8;color('black');text(tX,tY, 'GFLIB_Sign_FLT', 'horizontalAlignment', 'center');
  GFLIB_SinCos_FLT : Subsystem  TreatAsAtomicUnit=on  mask(GFLIB_SinCos_FLT){}
      mask help: Calculation of sine and cosine of the same argument in single precision floating-point implementation. Refer to the AMMCLIB User's Guide for further details.
      mask init: same as ammclib_bam_S32K3xx/GDFLIB/F16/GDFLIB_FilterFIR_F16
      settings: RTWSystemCode=Inline
      mask Help: web([fileparts(which('ammclib_bam_S32K3xx.slx')) '/../doc/S32K3XXMCLUG.pdf'], '-browser')
      mask Display: pos = get_param(gcb, 'Position');width = pos(3) - pos(1); height = pos(4) - pos(2);tX=width/2;tY=height - 8;color('black');text(tX,tY, 'GFLIB_SinCos_FLT', 'horizontalAlignment', 'center');
  GFLIB_Sin_FLT : Subsystem  TreatAsAtomicUnit=on  mask(GFLIB_Sin_FLT){}
      mask help: Sine function in single precision floating-point implementation. Refer to the AMMCLIB User's Guide for further details.
      mask init: same as ammclib_bam_S32K3xx/GDFLIB/F16/GDFLIB_FilterFIR_F16
      settings: RTWSystemCode=Inline
      mask Help: web([fileparts(which('ammclib_bam_S32K3xx.slx')) '/../doc/S32K3XXMCLUG.pdf'], '-browser')
      mask Display: pos = get_param(gcb, 'Position');width = pos(3) - pos(1); height = pos(4) - pos(2);tX=width/2;tY=height - 8;color('black');text(tX,tY, 'GFLIB_Sin_FLT', 'horizontalAlignment', 'center');
  GFLIB_Sqrt_FLT : Subsystem  TreatAsAtomicUnit=on  mask(GFLIB_Sqrt_FLT){}
      mask help: Square root approximation in single precision floating-point implementation. Refer to the AMMCLIB User's Guide for further details.
      mask init: same as ammclib_bam_S32K3xx/GDFLIB/F16/GDFLIB_FilterFIR_F16
      settings: RTWSystemCode=Inline
      mask Help: web([fileparts(which('ammclib_bam_S32K3xx.slx')) '/../doc/S32K3XXMCLUG.pdf'], '-browser')
      mask Display: pos = get_param(gcb, 'Position');width = pos(3) - pos(1); height = pos(4) - pos(2);tX=width/2;tY=height - 8;color('black');text(tX,tY, 'GFLIB_Sqrt_FLT', 'horizontalAlignment', 'center');
  GFLIB_Tan_FLT : Subsystem  TreatAsAtomicUnit=on  mask(GFLIB_Tan_FLT){}
      mask help: Tangent function in single precision floating-point implementation. Refer to the AMMCLIB User's Guide for further details.
      mask init: same as ammclib_bam_S32K3xx/GDFLIB/F16/GDFLIB_FilterFIR_F16
      settings: RTWSystemCode=Inline
      mask Help: web([fileparts(which('ammclib_bam_S32K3xx.slx')) '/../doc/S32K3XXMCLUG.pdf'], '-browser')
      mask Display: pos = get_param(gcb, 'Position');width = pos(3) - pos(1); height = pos(4) - pos(2);tX=width/2;tY=height - 8;color('black');text(tX,tY, 'GFLIB_Tan_FLT', 'horizontalAlignment', 'center');
  GFLIB_UpperLimit_FLT : Subsystem  TreatAsAtomicUnit=on  mask(GFLIB_UpperLimit_FLT){showStates=Hide (faster execution), fltUpperLimit=0}
      mask prompts: showStates "Show parameters as inputs:"; fltUpperLimit "fltUpperLimit (Value determining the upper limit threshold):"
      mask help: Upper limit function in single precision floating-point implementation. Refer to the AMMCLIB User's Guide for further details.
      mask init:
      | ddName = get_param(bdroot,'DataDictionary');
      | if length(ddName)==0
      |   set_param(bdroot,'DataDictionary','ammclib_types.sldd');
      | else
      |   dd = Simulink.data.dictionary.open(ddName);
      |   data = getSection(dd,'Design Data');
      |   if ~exist(data,'SWLIBS_2Syst_F16')
      |     addDataSource(dd,'ammclib_types.sldd');
      |     saveChanges(dd);
      |   end
      | end
      | 
      | if showStates == 1
      |   % hidden state variables
      |   if strcmp(get_param([gcb '/fltUpperLimit'], 'BlockType'), 'Inport')
      |     posblk = get_param(gcb, 'Position');
      | 
      |     pos = get_param([gcb, '/fltUpperLimit'], 'Position');
      |     orient = get_param([gcb, '/fltUpperLimit'], 'Orientation');
      |     delete_block([gcb, '/fltUpperLimit']);
      |     add_block('built-in/Ground', [gcb, '/fltUpperLimit'], 'Position', pos, 'Orientation', orient);
      | 
      | 
      |     set_param([gcb '/fltIn'], 'Port', '1');
      | 
      |     tmpOutCnt=0;
      |     tmpOutCnt=tmpOutCnt+1;
      |     set_param([gcb '/fltOut'], 'Port', num2str(tmpOutCnt));
      | 
      | set_param(gcb,'MaskEnables',{'on','on'});
      | 
      |     if (posblk(4) - posblk(2)) > 50
      |       height = 50;
      |       set_param(gcb,'Position',[posblk(1), posblk(2), posblk(3), posblk(2)+height])
      |     end
      |   end
      | else
      |   % shown state variables
      |   if strcmp(get_param([gcb '/fltUpperLimit'], 'BlockType'), 'Ground')
      |     posblk = get_param(gcb, 'Position');
      | 
      |     pos = get_param([gcb, '/fltUpperLimit'], 'Position');
      |     orient = get_param([gcb, '/fltUpperLimit'], 'Orientation');
      |     delete_block([gcb, '/fltUpperLimit']);
      |     add_block('built-in/Inport', [gcb, '/fltUpperLimit'], 'Position', pos, 'Orientation', orient, 'OutDataTypeStr', 'single');
      | 
      | 
      | 
      | 
      |     set_param([gcb '/fltIn'], 'Port', '1');
      |     set_param([gcb '/fltUpperLimit'], 'Port', '2');
      | 
      |     tmpOutCnt=0;
      |     tmpOutCnt=tmpOutCnt+1;
      |     set_param([gcb '/fltOut'], 'Port', num2str(tmpOutCnt));
      | 
      |     set_param(gcb,'MaskEnables',{'on','off'});
      | 
      |     if (posblk(4) - posblk(2)) < 75
      |       height = 75;
      |       set_param(gcb,'Position',[posblk(1), posblk(2), posblk(3), posblk(2)+height])
      |     end
      |   end
      | end
      settings: RTWSystemCode=Inline
      mask Help: web([fileparts(which('ammclib_bam_S32K3xx.slx')) '/../doc/S32K3XXMCLUG.pdf'], '-browser')
      mask TypeOptions showStates: Hide (faster execution) | Show (parameters can be changed during simulation)
      mask Callback showStates:
      | maskStr=get_param(gcb,'showStates');
      | if strcmp(maskStr,'Hide (faster execution)')
      |   if strcmp(get_param([gcb '/fltUpperLimit'], 'BlockType'), 'Inport')
      | set_param(gcb,'MaskEnables',{'on','on'});
      |   end
      | else
      |   if strcmp(get_param([gcb '/fltUpperLimit'], 'BlockType'), 'Ground')
      |     set_param(gcb,'MaskEnables',{'on','off'});
      |   end
      | end
      mask Display:
      | color('black');
      | pos = get_param(gcb, 'Position');
      | width = pos(3) - pos(1);
      | height = pos(4) - pos(2);
      | tX=width/2;
      | tY=height - 8;
      | color('black');
      | text(tX,tY, 'GFLIB_UpperLimit_FLT', 'horizontalAlignment', 'center');
      | if showStates == 2
      |   color('red');
      |   text(tX,tY - 20, ['debugging mode' char(13) char(10) '(limited performance)'], 'horizontalAlignment', 'center');
      | end
  GFLIB_VLog10_FLT : Subsystem  TreatAsAtomicUnit=on  mask(GFLIB_VLog10_FLT){}
      mask help: Single precision floating-point implementation of the GFLIB_VLog10 function, which computes base-10 logarithm of all elements of a vector. Refer to the AMMCLIB User's Guide for further details.
      mask init: same as ammclib_bam_S32K3xx/GDFLIB/F16/GDFLIB_FilterFIR_F16
      settings: RTWSystemCode=Inline
      mask Help: web([fileparts(which('ammclib_bam_S32K3xx.slx')) '/../doc/S32K3XXMCLUG.pdf'], '-browser')
      mask Display: pos = get_param(gcb, 'Position');width = pos(3) - pos(1); height = pos(4) - pos(2);tX=width/2;tY=height - 8;color('black');text(tX,tY, 'GFLIB_VLog10_FLT', 'horizontalAlignment', 'center');
  GFLIB_VMin_FLT : Subsystem  TreatAsAtomicUnit=on  mask(GFLIB_VMin_FLT){}
      mask help: Single precision floating-point implementation of the GFLIB_VMin function, which finds the index of a vector minimum. Refer to the AMMCLIB User's Guide for further details.
      mask init: same as ammclib_bam_S32K3xx/GDFLIB/F16/GDFLIB_FilterFIR_F16
      settings: RTWSystemCode=Inline
      mask Help: web([fileparts(which('ammclib_bam_S32K3xx.slx')) '/../doc/S32K3XXMCLUG.pdf'], '-browser')
      mask Display: pos = get_param(gcb, 'Position');width = pos(3) - pos(1); height = pos(4) - pos(2);tX=width/2;tY=height - 8;color('black');text(tX,tY, 'GFLIB_VMin_FLT', 'horizontalAlignment', 'center');
  GFLIB_VectorLimit_FLT : Subsystem  TreatAsAtomicUnit=on  mask(GFLIB_VectorLimit_FLT){showStates=Hide (faster execution), fltLimit=0}
      mask prompts: showStates "Show parameters as inputs:"; fltLimit "fltLimit (The maximum magnitude of the input 2-element vector):"
      mask help: Single precision floating-point implementation of the GFLIB_VectorLimit function which limits the magnitude of the input 2-element vector, keeping its direction unchanged. Refer to the AMMCLIB User's Guide for further details.
      mask init:
      | ddName = get_param(bdroot,'DataDictionary');
      | if length(ddName)==0
      |   set_param(bdroot,'DataDictionary','ammclib_types.sldd');
      | else
      |   dd = Simulink.data.dictionary.open(ddName);
      |   data = getSection(dd,'Design Data');
      |   if ~exist(data,'SWLIBS_2Syst_F16')
      |     addDataSource(dd,'ammclib_types.sldd');
      |     saveChanges(dd);
      |   end
      | end
      | 
      | if showStates == 1
      |   % hidden state variables
      |   if strcmp(get_param([gcb '/fltLimit'], 'BlockType'), 'Inport')
      |     posblk = get_param(gcb, 'Position');
      | 
      |     pos = get_param([gcb, '/fltLimit'], 'Position');
      |     orient = get_param([gcb, '/fltLimit'], 'Orientation');
      |     delete_block([gcb, '/fltLimit']);
      |     add_block('built-in/Ground', [gcb, '/fltLimit'], 'Position', pos, 'Orientation', orient);
      | 
      | 
      |     set_param([gcb '/pIn'], 'Port', '1');
      | 
      |     tmpOutCnt=0;
      |     tmpOutCnt=tmpOutCnt+1;
      |     set_param([gcb '/bFlag'], 'Port', num2str(tmpOutCnt));
      |     tmpOutCnt=tmpOutCnt+1;
      |     set_param([gcb '/pOut'], 'Port', num2str(tmpOutCnt));
      | 
      | set_param(gcb,'MaskEnables',{'on','on'});
      | 
      |     if (posblk(4) - posblk(2)) > 75
      |       height = 75;
      |       set_param(gcb,'Position',[posblk(1), posblk(2), posblk(3), posblk(2)+height])
      |     end
      |   end
      | else
      |   % shown state variables
      |   if strcmp(get_param([gcb '/fltLimit'], 'BlockType'), 'Ground')
      |     posblk = get_param(gcb, 'Position');
      | 
      |     pos = get_param([gcb, '/fltLimit'], 'Position');
      |     orient = get_param([gcb, '/fltLimit'], 'Orientation');
      |     delete_block([gcb, '/fltLimit']);
      |     add_block('built-in/Inport', [gcb, '/fltLimit'], 'Position', pos, 'Orientation', orient, 'OutDataTypeStr', 'single');
      | 
      | 
      | 
      | 
      |     set_param([gcb '/pIn'], 'Port', '1');
      |     set_param([gcb '/fltLimit'], 'Port', '2');
      | 
      |     tmpOutCnt=0;
      |     tmpOutCnt=tmpOutCnt+1;
      |     set_param([gcb '/bFlag'], 'Port', num2str(tmpOutCnt));
      |     tmpOutCnt=tmpOutCnt+1;
      |     set_param([gcb '/pOut'], 'Port', num2str(tmpOutCnt));
      | 
      |     set_param(gcb,'MaskEnables',{'on','off'});
      | 
      |     if (posblk(4) - posblk(2)) < 75
      |       height = 75;
      |       set_param(gcb,'Position',[posblk(1), posblk(2), posblk(3), posblk(2)+height])
      |     end
      |   end
      | end
      settings: RTWSystemCode=Inline
      mask Help: web([fileparts(which('ammclib_bam_S32K3xx.slx')) '/../doc/S32K3XXMCLUG.pdf'], '-browser')
      mask TypeOptions showStates: Hide (faster execution) | Show (parameters can be changed during simulation)
      mask Callback showStates:
      | maskStr=get_param(gcb,'showStates');
      | if strcmp(maskStr,'Hide (faster execution)')
      |   if strcmp(get_param([gcb '/fltLimit'], 'BlockType'), 'Inport')
      | set_param(gcb,'MaskEnables',{'on','on'});
      |   end
      | else
      |   if strcmp(get_param([gcb '/fltLimit'], 'BlockType'), 'Ground')
      |     set_param(gcb,'MaskEnables',{'on','off'});
      |   end
      | end
      mask Display:
      | color('black');
      | pos = get_param(gcb, 'Position');
      | width = pos(3) - pos(1);
      | height = pos(4) - pos(2);
      | tX=width/2;
      | tY=height - 8;
      | color('black');
      | text(tX,tY, 'GFLIB_VectorLimit_FLT', 'horizontalAlignment', 'center');
      | if showStates == 2
      |   color('red');
      |   text(tX,tY - 20, ['debugging mode' char(13) char(10) '(limited performance)'], 'horizontalAlignment', 'center');
      | end
